simulink model "model"  (R2014a)
(part 6 of 6)

  Pärnu_Jaagupi_haruliin_CN_35450914_110000_CN_35450919_110000/RConn3 -- T_35450919_110000;35000;10000_Audru_alajaam/LConn3 -- bus19/LConn1
  T_35394600_110000;35000;10000_Otepää_alajaam/LConn1 -- _CN_35394600_110000_CN_35420119_110000/LConn1
  T_35394600_110000;35000;10000_Otepää_alajaam/LConn2 -- _CN_35394600_110000_CN_35420119_110000/LConn2
  _CN_35394600_110000_CN_35420119_110000/LConn3 -- T_35394600_110000;35000;10000_Otepää_alajaam/LConn3 -- bus20/LConn1
  _CN_35394600_110000_CN_35420119_110000/RConn1 -- T_35420119_110000;15000;400_Elva_alajaam/LConn1 -- Maaritsa_—_Kanepi_110_kV_CN_35445333_110000_CN_35420119_110000/LConn1
  _CN_35394600_110000_CN_35420119_110000/RConn2 -- T_35420119_110000;15000;400_Elva_alajaam/LConn2 -- Maaritsa_—_Kanepi_110_kV_CN_35445333_110000_CN_35420119_110000/LConn2
  _CN_35394600_110000_CN_35420119_110000/RConn3 -- T_35420119_110000;15000;400_Elva_alajaam/LConn3 -- Maaritsa_—_Kanepi_110_kV_CN_35445333_110000_CN_35420119_110000/LConn3 -- bus21/LConn1
  Alutaguse_—_Estonia_Põhja_110_kV_CN_35367472_110000_CN_35594689_110000/LConn1 -- T_35367472_110000;35000;6000_Alutaguse_alajaam/LConn1 -- _CN_35367472_110000_CN_290177759_110000/LConn1 -- _CN_35367472_110000_CN_35451776_110000/LConn1 -- _CN_35367472_110000_CN_35451774_110000/LConn1 -- _CN_35367472_110000_CN_263282453_110000/LConn1 -- Kiikla_—_Alutaguse_110_kV_CN_35367472_110000_CN_263282454_110000/LConn1 -- Kiikla_—_Alutaguse_110_kV_CN_35367472_110000_CN_34920675_110000/RConn1 -- _CN_35367472_110000_CN_205980356_110000/RConn1 -- _CN_35367472_110000_CN_35367491_110000/LConn1 -- Alutaguse_—_Konsu_110_kV_CN_35367472_110000_CN_34903294_110000/LConn1
  Alutaguse_—_Estonia_Põhja_110_kV_CN_35367472_110000_CN_35594689_110000/LConn2 -- T_35367472_110000;35000;6000_Alutaguse_alajaam/LConn2 -- _CN_35367472_110000_CN_290177759_110000/LConn2 -- _CN_35367472_110000_CN_35451776_110000/LConn2 -- _CN_35367472_110000_CN_35451774_110000/LConn2 -- _CN_35367472_110000_CN_263282453_110000/LConn2 -- Kiikla_—_Alutaguse_110_kV_CN_35367472_110000_CN_263282454_110000/LConn2 -- Kiikla_—_Alutaguse_110_kV_CN_35367472_110000_CN_34920675_110000/RConn2 -- _CN_35367472_110000_CN_205980356_110000/RConn2 -- _CN_35367472_110000_CN_35367491_110000/LConn2 -- Alutaguse_—_Konsu_110_kV_CN_35367472_110000_CN_34903294_110000/LConn2
  Alutaguse_—_Estonia_Põhja_110_kV_CN_35367472_110000_CN_35594689_110000/LConn3 -- T_35367472_110000;35000;6000_Alutaguse_alajaam/LConn3 -- _CN_35367472_110000_CN_290177759_110000/LConn3 -- _CN_35367472_110000_CN_35451776_110000/LConn3 -- _CN_35367472_110000_CN_35451774_110000/LConn3 -- _CN_35367472_110000_CN_263282453_110000/LConn3 -- bus22/LConn1 -- Kiikla_—_Alutaguse_110_kV_CN_35367472_110000_CN_263282454_110000/LConn3 -- Kiikla_—_Alutaguse_110_kV_CN_35367472_110000_CN_34920675_110000/RConn3 -- _CN_35367472_110000_CN_205980356_110000/RConn3 -- _CN_35367472_110000_CN_35367491_110000/LConn3 -- Alutaguse_—_Konsu_110_kV_CN_35367472_110000_CN_34903294_110000/LConn3
  T_35594689__/LConn1 -- Alutaguse_—_Estonia_Põhja_110_kV_CN_35367472_110000_CN_35594689_110000/RConn1
  T_35594689__/LConn2 -- Alutaguse_—_Estonia_Põhja_110_kV_CN_35367472_110000_CN_35594689_110000/RConn2
  Alutaguse_—_Estonia_Põhja_110_kV_CN_35367472_110000_CN_35594689_110000/RConn3 -- T_35594689__/LConn3 -- bus23/LConn1
  T_34903294_110000;35000;6000_Konsu_alajaam/LConn1 -- Alutaguse_—_Konsu_110_kV_CN_35367472_110000_CN_34903294_110000/RConn1
  T_34903294_110000;35000;6000_Konsu_alajaam/LConn2 -- Alutaguse_—_Konsu_110_kV_CN_35367472_110000_CN_34903294_110000/RConn2
  Alutaguse_—_Konsu_110_kV_CN_35367472_110000_CN_34903294_110000/RConn3 -- T_34903294_110000;35000;6000_Konsu_alajaam/LConn3 -- bus24/LConn1
  T_263282454_110000;6000_Kiikla_alajaam/LConn1 -- Kiikla_—_Alutaguse_110_kV_CN_35367472_110000_CN_263282454_110000/RConn1
  T_263282454_110000;6000_Kiikla_alajaam/LConn2 -- Kiikla_—_Alutaguse_110_kV_CN_35367472_110000_CN_263282454_110000/RConn2
  Kiikla_—_Alutaguse_110_kV_CN_35367472_110000_CN_263282454_110000/RConn3 -- T_263282454_110000;6000_Kiikla_alajaam/LConn3 -- bus25/LConn1
  _CN_35367472_110000_CN_35367491_110000/RConn1 -- T_35367491_110000;35000;10000;6000_Aidu_alajaam/LConn1 -- Püssi_—_Aidu_110_kV_CN_35367491_110000_CN_34920713_110000/LConn1 -- Püssi_—_Aidu_110_kV_CN_35367491_110000_CN_34920699_110000/LConn1 -- _CN_35367491_110000_CN_35594719_110000/LConn1 -- Püssi_—_Aidu_110_kV_CN_35367491_110000_CN_34920675_110000/RConn1
  _CN_35367472_110000_CN_35367491_110000/RConn2 -- T_35367491_110000;35000;10000;6000_Aidu_alajaam/LConn2 -- Püssi_—_Aidu_110_kV_CN_35367491_110000_CN_34920713_110000/LConn2 -- Püssi_—_Aidu_110_kV_CN_35367491_110000_CN_34920699_110000/LConn2 -- _CN_35367491_110000_CN_35594719_110000/LConn2 -- Püssi_—_Aidu_110_kV_CN_35367491_110000_CN_34920675_110000/RConn2
  _CN_35367472_110000_CN_35367491_110000/RConn3 -- T_35367491_110000;35000;10000;6000_Aidu_alajaam/LConn3 -- Püssi_—_Aidu_110_kV_CN_35367491_110000_CN_34920713_110000/LConn3 -- Püssi_—_Aidu_110_kV_CN_35367491_110000_CN_34920699_110000/LConn3 -- bus26/LConn1 -- _CN_35367491_110000_CN_35594719_110000/LConn3 -- Püssi_—_Aidu_110_kV_CN_35367491_110000_CN_34920675_110000/RConn3
  T_290177759_110000_Illuka_alajaam/LConn1 -- _CN_35367472_110000_CN_290177759_110000/RConn1
  T_290177759_110000_Illuka_alajaam/LConn2 -- _CN_35367472_110000_CN_290177759_110000/RConn2
  _CN_35367472_110000_CN_290177759_110000/RConn3 -- T_290177759_110000_Illuka_alajaam/LConn3 -- bus27/LConn1
  _CN_35367472_110000_CN_35451776_110000/RConn1 -- T_35451776_110000;35000;15000;10000_Mustvee_alajaam/LConn1 -- Saare_—_Mustvee_110_kV_CN_35451776_110000_CN_180118919_110000/LConn1
  _CN_35367472_110000_CN_35451776_110000/RConn2 -- T_35451776_110000;35000;15000;10000_Mustvee_alajaam/LConn2 -- Saare_—_Mustvee_110_kV_CN_35451776_110000_CN_180118919_110000/LConn2
  _CN_35367472_110000_CN_35451776_110000/RConn3 -- T_35451776_110000;35000;15000;10000_Mustvee_alajaam/LConn3 -- Saare_—_Mustvee_110_kV_CN_35451776_110000_CN_180118919_110000/LConn3 -- bus28/LConn1
  _CN_35367472_110000_CN_35451774_110000/RConn1 -- T_35451774_110000;35000;15000;10000_Jõgeva_alajaam/LConn1 -- Jõgeva_—_Põdra_110_kV_CN_263282458_110000_CN_35451774_110000/LConn1
  _CN_35367472_110000_CN_35451774_110000/RConn2 -- T_35451774_110000;35000;15000;10000_Jõgeva_alajaam/LConn2 -- Jõgeva_—_Põdra_110_kV_CN_263282458_110000_CN_35451774_110000/LConn2
  _CN_35367472_110000_CN_35451774_110000/RConn3 -- T_35451774_110000;35000;15000;10000_Jõgeva_alajaam/LConn3 -- Jõgeva_—_Põdra_110_kV_CN_263282458_110000_CN_35451774_110000/LConn3 -- bus29/LConn1
  T_263282453_110000;10000_Kantküla_alajaam/LConn1 -- _CN_35367472_110000_CN_263282453_110000/RConn1
  T_263282453_110000;10000_Kantküla_alajaam/LConn2 -- _CN_35367472_110000_CN_263282453_110000/RConn2
  _CN_35367472_110000_CN_263282453_110000/RConn3 -- T_263282453_110000;10000_Kantküla_alajaam/LConn3 -- bus30/LConn1
  _CN_35022089_110000_CN_35022082_110000/LConn1 -- T_35022089_110000;35000;10000_Sikassaare_alajaam/LConn1 -- _CN_35022089_110000_CN_35022087_110000/LConn1 -- _CN_35022089_110000_CN_35022100_110000/LConn1
  _CN_35022089_110000_CN_35022082_110000/LConn2 -- T_35022089_110000;35000;10000_Sikassaare_alajaam/LConn2 -- _CN_35022089_110000_CN_35022087_110000/LConn2 -- _CN_35022089_110000_CN_35022100_110000/LConn2
  _CN_35022089_110000_CN_35022082_110000/LConn3 -- T_35022089_110000;35000;10000_Sikassaare_alajaam/LConn3 -- _CN_35022089_110000_CN_35022087_110000/LConn3 -- _CN_35022089_110000_CN_35022100_110000/LConn3 -- bus31/LConn1
  T_35022082_110000;10000_Orissaare_alajaam/LConn1 -- _CN_35022089_110000_CN_35022082_110000/RConn1
  T_35022082_110000;10000_Orissaare_alajaam/LConn2 -- _CN_35022089_110000_CN_35022082_110000/RConn2
  _CN_35022089_110000_CN_35022082_110000/RConn3 -- T_35022082_110000;10000_Orissaare_alajaam/LConn3 -- bus32/LConn1
  T_35022087_110000;10000_Valjala_alajaam/LConn1 -- _CN_35022089_110000_CN_35022087_110000/RConn1
  T_35022087_110000;10000_Valjala_alajaam/LConn2 -- _CN_35022089_110000_CN_35022087_110000/RConn2
  _CN_35022089_110000_CN_35022087_110000/RConn3 -- T_35022087_110000;10000_Valjala_alajaam/LConn3 -- bus33/LConn1
  T_35022100_110000;35000;10000_Leisi_alajaam/LConn1 -- _CN_35022089_110000_CN_35022100_110000/RConn1
  T_35022100_110000;35000;10000_Leisi_alajaam/LConn2 -- _CN_35022089_110000_CN_35022100_110000/RConn2
  _CN_35022089_110000_CN_35022100_110000/RConn3 -- T_35022100_110000;35000;10000_Leisi_alajaam/LConn3 -- bus34/LConn1
  T_35367481_110000_Allika_alajaam/LConn1 -- Balti_EJ_—_Allika_110_kV_CN_35367481_110000_CN_34682059_110000/RConn1
  T_35367481_110000_Allika_alajaam/LConn2 -- Balti_EJ_—_Allika_110_kV_CN_35367481_110000_CN_34682059_110000/RConn2
  Balti_EJ_—_Allika_110_kV_CN_35367481_110000_CN_34682059_110000/RConn3 -- T_35367481_110000_Allika_alajaam/LConn3 -- bus35/LConn1
  T_35451772_110000;15000_Suure_Jaani_alajaam/LConn1 -- Paide_—_Türi_—_Vändra_110_kV_CN_35450940_110000_CN_35451772_110000/RConn1
  T_35451772_110000;15000_Suure_Jaani_alajaam/LConn2 -- Paide_—_Türi_—_Vändra_110_kV_CN_35450940_110000_CN_35451772_110000/RConn2
  Paide_—_Türi_—_Vändra_110_kV_CN_35450940_110000_CN_35451772_110000/RConn3 -- T_35451772_110000;15000_Suure_Jaani_alajaam/LConn3 -- bus36/LConn1
  T_35451763_110000;35000;10000_Türi_alajaam/LConn1 -- Paide_—_Türi_—_Vändra_110_kV_CN_35450940_110000_CN_35451763_110000/RConn1
  T_35451763_110000;35000;10000_Türi_alajaam/LConn2 -- Paide_—_Türi_—_Vändra_110_kV_CN_35450940_110000_CN_35451763_110000/RConn2
  Paide_—_Türi_—_Vändra_110_kV_CN_35450940_110000_CN_35451763_110000/RConn3 -- T_35451763_110000;35000;10000_Türi_alajaam/LConn3 -- bus37/LConn1
  Paide_—_Türi_—_Vändra_110_kV_CN_35450940_110000_CN_35343343_110000/RConn1 -- T_35343343_330000;110000;35000;10000_Paide_alajaam/RConn1 -- Paide_—_Rapla_110_kV_CN_35343343_110000_CN_35379710_110000/LConn1 -- L_35343343/LConn1 -- _CN_34903268_110000_CN_35343343_110000/LConn1
  Paide_—_Türi_—_Vändra_110_kV_CN_35450940_110000_CN_35343343_110000/RConn2 -- T_35343343_330000;110000;35000;10000_Paide_alajaam/RConn2 -- Paide_—_Rapla_110_kV_CN_35343343_110000_CN_35379710_110000/LConn2 -- L_35343343/LConn2 -- _CN_34903268_110000_CN_35343343_110000/LConn2
  Paide_—_Türi_—_Vändra_110_kV_CN_35450940_110000_CN_35343343_110000/RConn3 -- T_35343343_330000;110000;35000;10000_Paide_alajaam/RConn3 -- Paide_—_Rapla_110_kV_CN_35343343_110000_CN_35379710_110000/LConn3 -- L_35343343/LConn3 -- bus38/LConn1 -- _CN_34903268_110000_CN_35343343_110000/LConn3
  T_35594719__/LConn1 -- _CN_35367491_110000_CN_35594719_110000/RConn1
  T_35594719__/LConn2 -- _CN_35367491_110000_CN_35594719_110000/RConn2
  _CN_35367491_110000_CN_35594719_110000/RConn3 -- T_35594719__/LConn3 -- bus39/LConn1
  T_34920713_110000;35000;10000_Väike_Maarja_alajaam/LConn1 -- Püssi_—_Aidu_110_kV_CN_35367491_110000_CN_34920713_110000/RConn1
  T_34920713_110000;35000;10000_Väike_Maarja_alajaam/LConn2 -- Püssi_—_Aidu_110_kV_CN_35367491_110000_CN_34920713_110000/RConn2
  Püssi_—_Aidu_110_kV_CN_35367491_110000_CN_34920713_110000/RConn3 -- T_34920713_110000;35000;10000_Väike_Maarja_alajaam/LConn3 -- bus40/LConn1
  Püssi_—_Aidu_110_kV_CN_35367491_110000_CN_34920699_110000/RConn1 -- T_34920699_330000;110000;35000;10000_Rakvere_alajaam/RConn1 -- Tapa_—_Rakvere_110_kV_CN_34920699_110000_CN_35384064_110000/RConn1 -- L_34920699/LConn1 -- _CN_34920702_110000_CN_34920699_110000/LConn1 -- Haljala_haruliin_CN_34920691_110000_CN_34920699_110000/LConn1
  Püssi_—_Aidu_110_kV_CN_35367491_110000_CN_34920699_110000/RConn2 -- T_34920699_330000;110000;35000;10000_Rakvere_alajaam/RConn2 -- Tapa_—_Rakvere_110_kV_CN_34920699_110000_CN_35384064_110000/RConn2 -- L_34920699/LConn2 -- _CN_34920702_110000_CN_34920699_110000/LConn2 -- Haljala_haruliin_CN_34920691_110000_CN_34920699_110000/LConn2
  Püssi_—_Aidu_110_kV_CN_35367491_110000_CN_34920699_110000/RConn3 -- T_34920699_330000;110000;35000;10000_Rakvere_alajaam/RConn3 -- Tapa_—_Rakvere_110_kV_CN_34920699_110000_CN_35384064_110000/RConn3 -- L_34920699/LConn3 -- bus41/LConn1 -- _CN_34920702_110000_CN_34920699_110000/LConn3 -- Haljala_haruliin_CN_34920691_110000_CN_34920699_110000/LConn3
  Kanepi_—_Võru_110_kV_CN_35445333_110000_CN_35445334_110000/LConn1 -- T_35445333__/LConn1 -- Maaritsa_—_Kanepi_110_kV_CN_35445333_110000_CN_35420117_110000/LConn1 -- Maaritsa_—_Kanepi_110_kV_CN_35445333_110000_CN_35420119_110000/RConn1 -- Maaritsa_—_Kanepi_110_kV_CN_35445333_110000_CN_262457166_110000/LConn1 -- Maaritsa_—_Kanepi_110_kV_CN_35445333_110000_CN_34682089_110000/LConn1
  Kanepi_—_Võru_110_kV_CN_35445333_110000_CN_35445334_110000/LConn2 -- T_35445333__/LConn2 -- Maaritsa_—_Kanepi_110_kV_CN_35445333_110000_CN_35420117_110000/LConn2 -- Maaritsa_—_Kanepi_110_kV_CN_35445333_110000_CN_35420119_110000/RConn2 -- Maaritsa_—_Kanepi_110_kV_CN_35445333_110000_CN_262457166_110000/LConn2 -- Maaritsa_—_Kanepi_110_kV_CN_35445333_110000_CN_34682089_110000/LConn2
  Kanepi_—_Võru_110_kV_CN_35445333_110000_CN_35445334_110000/LConn3 -- T_35445333__/LConn3 -- Maaritsa_—_Kanepi_110_kV_CN_35445333_110000_CN_35420117_110000/LConn3 -- Maaritsa_—_Kanepi_110_kV_CN_35445333_110000_CN_35420119_110000/RConn3 -- Maaritsa_—_Kanepi_110_kV_CN_35445333_110000_CN_262457166_110000/LConn3 -- Maaritsa_—_Kanepi_110_kV_CN_35445333_110000_CN_34682089_110000/LConn3 -- bus42/LConn1
  Kanepi_—_Võru_110_kV_CN_35445333_110000_CN_35445334_110000/RConn1 -- T_35445334_110000;35000;10000_Võru_alajaam/LConn1 -- Võru_—_Soo_110_kV_CN_35445334_110000_CN_35445340_110000/LConn1 -- Võru_—_Põlva_110_kV_CN_35445334_110000_CN_35594687_110000/LConn1 -- Võru_—_Põlva_110_kV_CN_35445334_110000_CN_35445343_110000/LConn1 -- _CN_35445334_110000_CN_182242759_110000/LConn1 -- _CN_35445334_110000_CN_34685113_110000/LConn1 -- _CN_35445334_110000_CN_35445335_110000/LConn1 -- _CN_35445334_110000_CN_182774903_110000/LConn1 -- _CN_35445334_110000_CN_263235177_110000/LConn1
  Kanepi_—_Võru_110_kV_CN_35445333_110000_CN_35445334_110000/RConn2 -- T_35445334_110000;35000;10000_Võru_alajaam/LConn2 -- Võru_—_Soo_110_kV_CN_35445334_110000_CN_35445340_110000/LConn2 -- Võru_—_Põlva_110_kV_CN_35445334_110000_CN_35594687_110000/LConn2 -- Võru_—_Põlva_110_kV_CN_35445334_110000_CN_35445343_110000/LConn2 -- _CN_35445334_110000_CN_182242759_110000/LConn2 -- _CN_35445334_110000_CN_34685113_110000/LConn2 -- _CN_35445334_110000_CN_35445335_110000/LConn2 -- _CN_35445334_110000_CN_182774903_110000/LConn2 -- _CN_35445334_110000_CN_263235177_110000/LConn2
  Kanepi_—_Võru_110_kV_CN_35445333_110000_CN_35445334_110000/RConn3 -- T_35445334_110000;35000;10000_Võru_alajaam/LConn3 -- Võru_—_Soo_110_kV_CN_35445334_110000_CN_35445340_110000/LConn3 -- Võru_—_Põlva_110_kV_CN_35445334_110000_CN_35594687_110000/LConn3 -- Võru_—_Põlva_110_kV_CN_35445334_110000_CN_35445343_110000/LConn3 -- _CN_35445334_110000_CN_182242759_110000/LConn3 -- _CN_35445334_110000_CN_34685113_110000/LConn3 -- _CN_35445334_110000_CN_35445335_110000/LConn3 -- _CN_35445334_110000_CN_182774903_110000/LConn3 -- _CN_35445334_110000_CN_263235177_110000/LConn3 -- bus43/LConn1
  T_35420117_110000;10000_Maaritsa_alajaam/LConn1 -- Maaritsa_—_Kanepi_110_kV_CN_35445333_110000_CN_35420117_110000/RConn1
  T_35420117_110000;10000_Maaritsa_alajaam/LConn2 -- Maaritsa_—_Kanepi_110_kV_CN_35445333_110000_CN_35420117_110000/RConn2
  Maaritsa_—_Kanepi_110_kV_CN_35445333_110000_CN_35420117_110000/RConn3 -- T_35420117_110000;10000_Maaritsa_alajaam/LConn3 -- bus44/LConn1
  Maaritsa_—_Kanepi_110_kV_CN_35445333_110000_CN_262457166_110000/RConn1 -- T_262457166_110000;35000;15000;10000_Rõngu_alajaam/LConn1 -- Rõngu_—_Tõrva_110_kV_CN_35445348_110000_CN_262457166_110000/LConn1
  Maaritsa_—_Kanepi_110_kV_CN_35445333_110000_CN_262457166_110000/RConn2 -- T_262457166_110000;35000;15000;10000_Rõngu_alajaam/LConn2 -- Rõngu_—_Tõrva_110_kV_CN_35445348_110000_CN_262457166_110000/LConn2
  Maaritsa_—_Kanepi_110_kV_CN_35445333_110000_CN_262457166_110000/RConn3 -- T_262457166_110000;35000;15000;10000_Rõngu_alajaam/LConn3 -- Rõngu_—_Tõrva_110_kV_CN_35445348_110000_CN_262457166_110000/LConn3 -- bus45/LConn1
  Maaritsa_—_Kanepi_110_kV_CN_35445333_110000_CN_34682089_110000/RConn1 -- T_34682089_330000;110000;35000;15000;10000_Tartu_alajaam/RConn1 -- Voldi_haruliin_CN_101153487_110000_CN_34682089_110000/LConn1 -- Tartu_—_Anne_&_Tartu_—_Tööstuse_110_kV_CN_34682089_110000_CN_30228363_110000/LConn1 -- Tartu_—_Emajõe_110_kV_CN_34682089_110000_CN_30222062_110000/LConn1 -- L_34682089/LConn1
  Maaritsa_—_Kanepi_110_kV_CN_35445333_110000_CN_34682089_110000/RConn2 -- T_34682089_330000;110000;35000;15000;10000_Tartu_alajaam/RConn2 -- Voldi_haruliin_CN_101153487_110000_CN_34682089_110000/LConn2 -- Tartu_—_Anne_&_Tartu_—_Tööstuse_110_kV_CN_34682089_110000_CN_30228363_110000/LConn2 -- Tartu_—_Emajõe_110_kV_CN_34682089_110000_CN_30222062_110000/LConn2 -- L_34682089/LConn2
  Maaritsa_—_Kanepi_110_kV_CN_35445333_110000_CN_34682089_110000/RConn3 -- T_34682089_330000;110000;35000;15000;10000_Tartu_alajaam/RConn3 -- Voldi_haruliin_CN_101153487_110000_CN_34682089_110000/LConn3 -- Tartu_—_Anne_&_Tartu_—_Tööstuse_110_kV_CN_34682089_110000_CN_30228363_110000/LConn3 -- Tartu_—_Emajõe_110_kV_CN_34682089_110000_CN_30222062_110000/LConn3 -- L_34682089/LConn3 -- bus46/LConn1
  T_35445340_110000;10000_Soo_alajaam/LConn1 -- Võru_—_Soo_110_kV_CN_35445334_110000_CN_35445340_110000/RConn1
  T_35445340_110000;10000_Soo_alajaam/LConn2 -- Võru_—_Soo_110_kV_CN_35445334_110000_CN_35445340_110000/RConn2
  Võru_—_Soo_110_kV_CN_35445334_110000_CN_35445340_110000/RConn3 -- T_35445340_110000;10000_Soo_alajaam/LConn3 -- bus47/LConn1
  T_35594687_110000;10000_Ruusa_alajaam/LConn1 -- Võru_—_Põlva_110_kV_CN_35445334_110000_CN_35594687_110000/RConn1
  T_35594687_110000;10000_Ruusa_alajaam/LConn2 -- Võru_—_Põlva_110_kV_CN_35445334_110000_CN_35594687_110000/RConn2
  Võru_—_Põlva_110_kV_CN_35445334_110000_CN_35594687_110000/RConn3 -- T_35594687_110000;10000_Ruusa_alajaam/LConn3 -- bus48/LConn1
  Võru_—_Põlva_110_kV_CN_35445334_110000_CN_35445343_110000/RConn1 -- T_35445343__Põlva_alajaam/LConn1 -- Kuuste_—_Põlva_110_kV_CN_35445343_110000_CN_35445346_110000/LConn1
  Võru_—_Põlva_110_kV_CN_35445334_110000_CN_35445343_110000/RConn2 -- T_35445343__Põlva_alajaam/LConn2 -- Kuuste_—_Põlva_110_kV_CN_35445343_110000_CN_35445346_110000/LConn2
  Võru_—_Põlva_110_kV_CN_35445334_110000_CN_35445343_110000/RConn3 -- T_35445343__Põlva_alajaam/LConn3 -- Kuuste_—_Põlva_110_kV_CN_35445343_110000_CN_35445346_110000/LConn3 -- bus49/LConn1
  _CN_35445334_110000_CN_182242759_110000/RConn1 -- T_182242759_110000;10000_Rõuge_alajaam/LConn1 -- _CN_263253461_110000_CN_182242759_110000/LConn1
  _CN_35445334_110000_CN_182242759_110000/RConn2 -- T_182242759_110000;10000_Rõuge_alajaam/LConn2 -- _CN_263253461_110000_CN_182242759_110000/LConn2
  _CN_35445334_110000_CN_182242759_110000/RConn3 -- T_182242759_110000;10000_Rõuge_alajaam/LConn3 -- _CN_263253461_110000_CN_182242759_110000/LConn3 -- bus50/LConn1
  _CN_35445334_110000_CN_34685113_110000/RConn1 -- T_34685113_330000;110000;35000;10000_Tsinguliina_alajaam/RConn1 -- Tsirguliina_—_Tõrva_110_kV_CN_35445348_110000_CN_34685113_110000/LConn1 -- _CN_34685113_110000_CN_35450869_110000/LConn1 -- L_34685113/LConn1
  _CN_35445334_110000_CN_34685113_110000/RConn2 -- T_34685113_330000;110000;35000;10000_Tsinguliina_alajaam/RConn2 -- Tsirguliina_—_Tõrva_110_kV_CN_35445348_110000_CN_34685113_110000/LConn2 -- _CN_34685113_110000_CN_35450869_110000/LConn2 -- L_34685113/LConn2
  _CN_35445334_110000_CN_34685113_110000/RConn3 -- T_34685113_330000;110000;35000;10000_Tsinguliina_alajaam/RConn3 -- Tsirguliina_—_Tõrva_110_kV_CN_35445348_110000_CN_34685113_110000/LConn3 -- _CN_34685113_110000_CN_35450869_110000/LConn3 -- L_34685113/LConn3 -- bus51/LConn1
  T_35445335_110000;35000;10000_Mõniste_alajaam/LConn1 -- _CN_35445334_110000_CN_35445335_110000/RConn1
  T_35445335_110000;35000;10000_Mõniste_alajaam/LConn2 -- _CN_35445334_110000_CN_35445335_110000/RConn2
  _CN_35445334_110000_CN_35445335_110000/RConn3 -- T_35445335_110000;35000;10000_Mõniste_alajaam/LConn3 -- bus52/LConn1
  T_182774903_110000;10000_Linda_alajaam/LConn1 -- _CN_35445334_110000_CN_182774903_110000/RConn1
  T_182774903_110000;10000_Linda_alajaam/LConn2 -- _CN_35445334_110000_CN_182774903_110000/RConn2
  _CN_35445334_110000_CN_182774903_110000/RConn3 -- T_182774903_110000;10000_Linda_alajaam/LConn3 -- bus53/LConn1
  T_263235177_110000;10000_Sõmerpalu_alajaam/LConn1 -- _CN_35445334_110000_CN_263235177_110000/RConn1
  T_263235177_110000;10000_Sõmerpalu_alajaam/LConn2 -- _CN_35445334_110000_CN_263235177_110000/RConn2
  _CN_35445334_110000_CN_263235177_110000/RConn3 -- T_263235177_110000;10000_Sõmerpalu_alajaam/LConn3 -- bus54/LConn1
  Kuuste_—_Põlva_110_kV_CN_35445343_110000_CN_35445346_110000/RConn1 -- T_35445346_110000;10000_Kuuste_alajaam/LConn1 -- Anne_—_Kuuste_110_kV_CN_35445346_110000_CN_30228363_110000/LConn1 -- Anne_—_Kuuste_110_kV_CN_35445346_110000_CN_35594688_110000/LConn1
  Kuuste_—_Põlva_110_kV_CN_35445343_110000_CN_35445346_110000/RConn2 -- T_35445346_110000;10000_Kuuste_alajaam/LConn2 -- Anne_—_Kuuste_110_kV_CN_35445346_110000_CN_30228363_110000/LConn2 -- Anne_—_Kuuste_110_kV_CN_35445346_110000_CN_35594688_110000/LConn2
  Kuuste_—_Põlva_110_kV_CN_35445343_110000_CN_35445346_110000/RConn3 -- T_35445346_110000;10000_Kuuste_alajaam/LConn3 -- Anne_—_Kuuste_110_kV_CN_35445346_110000_CN_30228363_110000/LConn3 -- Anne_—_Kuuste_110_kV_CN_35445346_110000_CN_35594688_110000/LConn3 -- bus55/LConn1
  Anne_—_Kuuste_110_kV_CN_35445346_110000_CN_30228363_110000/RConn1 -- T_30228363_110000;35000;15000;10000_Anne_alajaam/LConn1 -- Tartu_—_Anne_&_Tartu_—_Tööstuse_110_kV_CN_34682089_110000_CN_30228363_110000/RConn1
  Anne_—_Kuuste_110_kV_CN_35445346_110000_CN_30228363_110000/RConn2 -- T_30228363_110000;35000;15000;10000_Anne_alajaam/LConn2 -- Tartu_—_Anne_&_Tartu_—_Tööstuse_110_kV_CN_34682089_110000_CN_30228363_110000/RConn2
  Anne_—_Kuuste_110_kV_CN_35445346_110000_CN_30228363_110000/RConn3 -- T_30228363_110000;35000;15000;10000_Anne_alajaam/LConn3 -- Tartu_—_Anne_&_Tartu_—_Tööstuse_110_kV_CN_34682089_110000_CN_30228363_110000/RConn3 -- bus56/LConn1
  T_35594688_110000;15000_Alatskivi_alajaam/LConn1 -- Anne_—_Kuuste_110_kV_CN_35445346_110000_CN_35594688_110000/RConn1
  T_35594688_110000;15000_Alatskivi_alajaam/LConn2 -- Anne_—_Kuuste_110_kV_CN_35445346_110000_CN_35594688_110000/RConn2
  Anne_—_Kuuste_110_kV_CN_35445346_110000_CN_35594688_110000/RConn3 -- T_35594688_110000;15000_Alatskivi_alajaam/LConn3 -- bus57/LConn1
  Rõngu_—_Tõrva_110_kV_CN_35445348_110000_CN_262457166_110000/RConn1 -- T_35445348_110000;15000_Tõrva_alajaam/LConn1 -- Tõrva_—_Abja_110_kV_CN_35445348_110000_CN_35450872_110000/LConn1 -- Tsirguliina_—_Tõrva_110_kV_CN_35445348_110000_CN_34685113_110000/RConn1 -- Tsirguliina_—_Tõrva_110_kV_CN_35445348_110000_CN_35450869_110000/LConn1
  Rõngu_—_Tõrva_110_kV_CN_35445348_110000_CN_262457166_110000/RConn2 -- T_35445348_110000;15000_Tõrva_alajaam/LConn2 -- Tõrva_—_Abja_110_kV_CN_35445348_110000_CN_35450872_110000/LConn2 -- Tsirguliina_—_Tõrva_110_kV_CN_35445348_110000_CN_34685113_110000/RConn2 -- Tsirguliina_—_Tõrva_110_kV_CN_35445348_110000_CN_35450869_110000/LConn2
  Rõngu_—_Tõrva_110_kV_CN_35445348_110000_CN_262457166_110000/RConn3 -- T_35445348_110000;15000_Tõrva_alajaam/LConn3 -- Tõrva_—_Abja_110_kV_CN_35445348_110000_CN_35450872_110000/LConn3 -- Tsirguliina_—_Tõrva_110_kV_CN_35445348_110000_CN_34685113_110000/RConn3 -- Tsirguliina_—_Tõrva_110_kV_CN_35445348_110000_CN_35450869_110000/LConn3 -- bus58/LConn1
  T_35450872_110000;15000_Abja_alajaam/LConn1 -- Tõrva_—_Abja_110_kV_CN_35445348_110000_CN_35450872_110000/RConn1
  T_35450872_110000;15000_Abja_alajaam/LConn2 -- Tõrva_—_Abja_110_kV_CN_35445348_110000_CN_35450872_110000/RConn2
  Tõrva_—_Abja_110_kV_CN_35445348_110000_CN_35450872_110000/RConn3 -- T_35450872_110000;15000_Abja_alajaam/LConn3 -- bus59/LConn1
  Tsirguliina_—_Tõrva_110_kV_CN_35445348_110000_CN_35450869_110000/RConn1 -- T_35450869_110000;10000_Valga_alajaam/LConn1 -- _CN_34685113_110000_CN_35450869_110000/RConn1
  Tsirguliina_—_Tõrva_110_kV_CN_35445348_110000_CN_35450869_110000/RConn2 -- T_35450869_110000;10000_Valga_alajaam/LConn2 -- _CN_34685113_110000_CN_35450869_110000/RConn2
  Tsirguliina_—_Tõrva_110_kV_CN_35445348_110000_CN_35450869_110000/RConn3 -- T_35450869_110000;10000_Valga_alajaam/LConn3 -- _CN_34685113_110000_CN_35450869_110000/RConn3 -- bus60/LConn1
  Kiisa_—_Keila_110_kV_CN_34935436_110000_CN_262229346_110000/LConn1 -- T_34935436_330000;220000;110000;35000;10000_Kiisa_alajaam/RConn1 -- _CN_34935436_110000_CN_265791084_110000/LConn1 -- L_34935436/LConn1 -- Kiisa_—_Järve_110_kV_CN_34935436_110000_CN_34968246_110000/LConn1 -- Kiisa_—_Järve_110_kV_CN_34935436_110000_CN_34968285_110000/LConn1 -- Kiisa_—_Ellamaa_CN_34935436_110000_CN_35379710_110000/LConn1 -- Kiisa_—_Ellamaa_CN_34935436_110000_CN_34988535_110000/LConn1 -- Kiisa_—_Ellamaa_CN_34935436_110000_CN_34988502_110000/LConn1 -- Harku_—_Kiisa_110_kV_CN_34935436_110000_CN_34968224_110000/LConn1 -- Kiisa_—_Laagri_110_kV_CN_34935436_110000_CN_34988471_110000/LConn1 -- Kiisa_—_Laagri_110_kV_CN_34935436_110000_CN_34935452_110000/LConn1
  Kiisa_—_Keila_110_kV_CN_34935436_110000_CN_262229346_110000/LConn2 -- T_34935436_330000;220000;110000;35000;10000_Kiisa_alajaam/RConn2 -- _CN_34935436_110000_CN_265791084_110000/LConn2 -- L_34935436/LConn2 -- Kiisa_—_Järve_110_kV_CN_34935436_110000_CN_34968246_110000/LConn2 -- Kiisa_—_Järve_110_kV_CN_34935436_110000_CN_34968285_110000/LConn2 -- Kiisa_—_Ellamaa_CN_34935436_110000_CN_35379710_110000/LConn2 -- Kiisa_—_Ellamaa_CN_34935436_110000_CN_34988535_110000/LConn2 -- Kiisa_—_Ellamaa_CN_34935436_110000_CN_34988502_110000/LConn2 -- Harku_—_Kiisa_110_kV_CN_34935436_110000_CN_34968224_110000/LConn2 -- Kiisa_—_Laagri_110_kV_CN_34935436_110000_CN_34988471_110000/LConn2 -- Kiisa_—_Laagri_110_kV_CN_34935436_110000_CN_34935452_110000/LConn2
  Kiisa_—_Keila_110_kV_CN_34935436_110000_CN_262229346_110000/LConn3 -- T_34935436_330000;220000;110000;35000;10000_Kiisa_alajaam/RConn3 -- _CN_34935436_110000_CN_265791084_110000/LConn3 -- L_34935436/LConn3 -- bus61/LConn1 -- Kiisa_—_Järve_110_kV_CN_34935436_110000_CN_34968246_110000/LConn3 -- Kiisa_—_Järve_110_kV_CN_34935436_110000_CN_34968285_110000/LConn3 -- Kiisa_—_Ellamaa_CN_34935436_110000_CN_35379710_110000/LConn3 -- Kiisa_—_Ellamaa_CN_34935436_110000_CN_34988535_110000/LConn3 -- Kiisa_—_Ellamaa_CN_34935436_110000_CN_34988502_110000/LConn3 -- Harku_—_Kiisa_110_kV_CN_34935436_110000_CN_34968224_110000/LConn3 -- Kiisa_—_Laagri_110_kV_CN_34935436_110000_CN_34988471_110000/LConn3 -- Kiisa_—_Laagri_110_kV_CN_34935436_110000_CN_34935452_110000/LConn3
  Kiisa_—_Keila_110_kV_CN_34935436_110000_CN_262229346_110000/RConn1 -- T_262229346_110000;35000;10000_Keila_alajaam/LConn1 -- Keila_—_Paldiski_110_kV_CN_35550404_110000_CN_262229346_110000/LConn1 -- Keila_—_Rummu_110_kV_CN_262229346_110000_CN_34988486_110000/LConn1 -- Harku_—_Keila_110_kV_CN_34968224_110000_CN_262229346_110000/LConn1
  Kiisa_—_Keila_110_kV_CN_34935436_110000_CN_262229346_110000/RConn2 -- T_262229346_110000;35000;10000_Keila_alajaam/LConn2 -- Keila_—_Paldiski_110_kV_CN_35550404_110000_CN_262229346_110000/LConn2 -- Keila_—_Rummu_110_kV_CN_262229346_110000_CN_34988486_110000/LConn2 -- Harku_—_Keila_110_kV_CN_34968224_110000_CN_262229346_110000/LConn2
  Kiisa_—_Keila_110_kV_CN_34935436_110000_CN_262229346_110000/RConn3 -- T_262229346_110000;35000;10000_Keila_alajaam/LConn3 -- Keila_—_Paldiski_110_kV_CN_35550404_110000_CN_262229346_110000/LConn3 -- Keila_—_Rummu_110_kV_CN_262229346_110000_CN_34988486_110000/LConn3 -- bus62/LConn1 -- Harku_—_Keila_110_kV_CN_34968224_110000_CN_262229346_110000/LConn3
  Kiisa_—_Järve_110_kV_CN_34935436_110000_CN_34968246_110000/RConn1 -- T_34968246_110000;10000;6000_Järve_alajaam/LConn1 -- Järve_—_Ülemiste_110_kV_CN_34968246_110000_CN_34968248_110000/LConn1 -- Iru_—_Järve_&_Järveküla_—_Järve_110_kV_CN_34968246_110000_CN_34968251_110000/LConn1 -- Iru_—_Järve_&_Järveküla_—_Järve_110_kV_CN_34968246_110000_CN_72668114_110000/LConn1
  Kiisa_—_Järve_110_kV_CN_34935436_110000_CN_34968246_110000/RConn2 -- T_34968246_110000;10000;6000_Järve_alajaam/LConn2 -- Järve_—_Ülemiste_110_kV_CN_34968246_110000_CN_34968248_110000/LConn2 -- Iru_—_Järve_&_Järveküla_—_Järve_110_kV_CN_34968246_110000_CN_34968251_110000/LConn2 -- Iru_—_Järve_&_Järveküla_—_Järve_110_kV_CN_34968246_110000_CN_72668114_110000/LConn2
  Kiisa_—_Järve_110_kV_CN_34935436_110000_CN_34968246_110000/RConn3 -- T_34968246_110000;10000;6000_Järve_alajaam/LConn3 -- Järve_—_Ülemiste_110_kV_CN_34968246_110000_CN_34968248_110000/LConn3 -- Iru_—_Järve_&_Järveküla_—_Järve_110_kV_CN_34968246_110000_CN_34968251_110000/LConn3 -- Iru_—_Järve_&_Järveküla_—_Järve_110_kV_CN_34968246_110000_CN_72668114_110000/LConn3 -- bus63/LConn1
  Kiisa_—_Järve_110_kV_CN_34935436_110000_CN_34968285_110000/RConn1 -- T_34968285_110000;10000_Jüri_alajaam/LConn1 -- Aruküla_—_Jüri_110_kV_CN_34968285_110000_CN_204914596_110000/RConn1
  Kiisa_—_Järve_110_kV_CN_34935436_110000_CN_34968285_110000/RConn2 -- T_34968285_110000;10000_Jüri_alajaam/LConn2 -- Aruküla_—_Jüri_110_kV_CN_34968285_110000_CN_204914596_110000/RConn2
  Kiisa_—_Järve_110_kV_CN_34935436_110000_CN_34968285_110000/RConn3 -- T_34968285_110000;10000_Jüri_alajaam/LConn3 -- Aruküla_—_Jüri_110_kV_CN_34968285_110000_CN_204914596_110000/RConn3 -- bus64/LConn1
  Kiisa_—_Ellamaa_CN_34935436_110000_CN_35379710_110000/RConn1 -- T_35379710_110000;10000_Kohila_alajaam/LConn1 -- Paide_—_Rapla_110_kV_CN_35343343_110000_CN_35379710_110000/RConn1
  Kiisa_—_Ellamaa_CN_34935436_110000_CN_35379710_110000/RConn2 -- T_35379710_110000;10000_Kohila_alajaam/LConn2 -- Paide_—_Rapla_110_kV_CN_35343343_110000_CN_35379710_110000/RConn2
  Kiisa_—_Ellamaa_CN_34935436_110000_CN_35379710_110000/RConn3 -- T_35379710_110000;10000_Kohila_alajaam/LConn3 -- Paide_—_Rapla_110_kV_CN_35343343_110000_CN_35379710_110000/RConn3 -- bus65/LConn1
  T_34988535_110000;35000;10000;6000_Ellamaa_alajaam/LConn1 -- Kiisa_—_Ellamaa_CN_34935436_110000_CN_34988535_110000/RConn1
  T_34988535_110000;35000;10000;6000_Ellamaa_alajaam/LConn2 -- Kiisa_—_Ellamaa_CN_34935436_110000_CN_34988535_110000/RConn2
  Kiisa_—_Ellamaa_CN_34935436_110000_CN_34988535_110000/RConn3 -- T_34988535_110000;35000;10000;6000_Ellamaa_alajaam/LConn3 -- bus66/LConn1
  Kiisa_—_Ellamaa_CN_34935436_110000_CN_34988502_110000/RConn1 -- T_34988502_110000;35000;10000_Risti_alajaam/LConn1 -- Lihula_—_Vigala_110_kV_CN_262755193_110000_CN_34988502_110000/LConn1
  Kiisa_—_Ellamaa_CN_34935436_110000_CN_34988502_110000/RConn2 -- T_34988502_110000;35000;10000_Risti_alajaam/LConn2 -- Lihula_—_Vigala_110_kV_CN_262755193_110000_CN_34988502_110000/LConn2
  Kiisa_—_Ellamaa_CN_34935436_110000_CN_34988502_110000/RConn3 -- T_34988502_110000;35000;10000_Risti_alajaam/LConn3 -- Lihula_—_Vigala_110_kV_CN_262755193_110000_CN_34988502_110000/LConn3 -- bus67/LConn1
  Harku_—_Kiisa_110_kV_CN_34935436_110000_CN_34968224_110000/RConn1 -- T_34968224_330000;110000;20000_Harku_ajajaam/RConn1 -- Harku_—_Veskimetsa_110_kV_CN_34968224_110000_CN_99350295_110000/LConn1 -- _CN_34968224_110000_CN_99369449_110000/LConn1 -- Harku_—_Keila_110_kV_CN_34968224_110000_CN_262229346_110000/RConn1 -- Harku_—_Keila_110_kV_CN_34968224_110000_CN_34988480_110000/LConn1 -- L_34968224/LConn1
  Harku_—_Kiisa_110_kV_CN_34935436_110000_CN_34968224_110000/RConn2 -- T_34968224_330000;110000;20000_Harku_ajajaam/RConn2 -- Harku_—_Veskimetsa_110_kV_CN_34968224_110000_CN_99350295_110000/LConn2 -- _CN_34968224_110000_CN_99369449_110000/LConn2 -- Harku_—_Keila_110_kV_CN_34968224_110000_CN_262229346_110000/RConn2 -- Harku_—_Keila_110_kV_CN_34968224_110000_CN_34988480_110000/LConn2 -- L_34968224/LConn2
  Harku_—_Kiisa_110_kV_CN_34935436_110000_CN_34968224_110000/RConn3 -- T_34968224_330000;110000;20000_Harku_ajajaam/RConn3 -- Harku_—_Veskimetsa_110_kV_CN_34968224_110000_CN_99350295_110000/LConn3 -- _CN_34968224_110000_CN_99369449_110000/LConn3 -- Harku_—_Keila_110_kV_CN_34968224_110000_CN_262229346_110000/RConn3 -- Harku_—_Keila_110_kV_CN_34968224_110000_CN_34988480_110000/LConn3 -- L_34968224/LConn3 -- bus68/LConn1
  T_34988471_110000;10000_Topi_alajaam/LConn1 -- Kiisa_—_Laagri_110_kV_CN_34935436_110000_CN_34988471_110000/RConn1
  T_34988471_110000;10000_Topi_alajaam/LConn2 -- Kiisa_—_Laagri_110_kV_CN_34935436_110000_CN_34988471_110000/RConn2
  Kiisa_—_Laagri_110_kV_CN_34935436_110000_CN_34988471_110000/RConn3 -- T_34988471_110000;10000_Topi_alajaam/LConn3 -- bus69/LConn1
  T_34935452_110000;35000;10000_Laagri_alajaam/LConn1 -- Kiisa_—_Laagri_110_kV_CN_34935436_110000_CN_34935452_110000/RConn1
  T_34935452_110000;35000;10000_Laagri_alajaam/LConn2 -- Kiisa_—_Laagri_110_kV_CN_34935436_110000_CN_34935452_110000/RConn2
  Kiisa_—_Laagri_110_kV_CN_34935436_110000_CN_34935452_110000/RConn3 -- T_34935452_110000;35000;10000_Laagri_alajaam/LConn3 -- bus70/LConn1
  _CN_34935436_110000_CN_265791084_110000/RConn1 -- G_265791084_Kiisa_AREJ/RConn1 -- _CN_34935436_330000_CN_265791084_110000/LConn1
  _CN_34935436_110000_CN_265791084_110000/RConn2 -- G_265791084_Kiisa_AREJ/RConn2 -- _CN_34935436_330000_CN_265791084_110000/LConn2
  _CN_34935436_110000_CN_265791084_110000/RConn3 -- G_265791084_Kiisa_AREJ/RConn3 -- _CN_34935436_330000_CN_265791084_110000/LConn3 -- bus71/LConn1
  T_34920702_110000;35000;10000_Rakvere_Põhja_alajaam/LConn1 -- _CN_34920702_110000_CN_34920699_110000/RConn1
  T_34920702_110000;35000;10000_Rakvere_Põhja_alajaam/LConn2 -- _CN_34920702_110000_CN_34920699_110000/RConn2
  _CN_34920702_110000_CN_34920699_110000/RConn3 -- T_34920702_110000;35000;10000_Rakvere_Põhja_alajaam/LConn3 -- bus72/LConn1
  T_29595798_110000;35000;10000_Loo_alajaam/LConn1 -- _CN_29595798_110000_CN_204914596_110000/RConn1
  T_29595798_110000;35000;10000_Loo_alajaam/LConn2 -- _CN_29595798_110000_CN_204914596_110000/RConn2
  _CN_29595798_110000_CN_204914596_110000/RConn3 -- T_29595798_110000;35000;10000_Loo_alajaam/LConn3 -- bus73/LConn1
  Harku_—_Veskimetsa_110_kV_CN_34968224_110000_CN_99350295_110000/RConn1 -- T_99350295_110000;35000;10000;6000_Veskimetsa_alajaam/LConn1 -- Kopli_—_Paljassaare_110_kV_CN_34968238_110000_CN_99350295_110000/LConn1
  Harku_—_Veskimetsa_110_kV_CN_34968224_110000_CN_99350295_110000/RConn2 -- T_99350295_110000;35000;10000;6000_Veskimetsa_alajaam/LConn2 -- Kopli_—_Paljassaare_110_kV_CN_34968238_110000_CN_99350295_110000/LConn2
  Harku_—_Veskimetsa_110_kV_CN_34968224_110000_CN_99350295_110000/RConn3 -- T_99350295_110000;35000;10000;6000_Veskimetsa_alajaam/LConn3 -- Kopli_—_Paljassaare_110_kV_CN_34968238_110000_CN_99350295_110000/LConn3 -- bus74/LConn1
  T_99369449__Kadaka_alajaam/LConn1 -- _CN_34968224_110000_CN_99369449_110000/RConn1
  T_99369449__Kadaka_alajaam/LConn2 -- _CN_34968224_110000_CN_99369449_110000/RConn2
  _CN_34968224_110000_CN_99369449_110000/RConn3 -- T_99369449__Kadaka_alajaam/LConn3 -- bus75/LConn1
  T_34988480_110000;10000_Tabasalu_alajaam/LConn1 -- Harku_—_Keila_110_kV_CN_34968224_110000_CN_34988480_110000/RConn1
  T_34988480_110000;10000_Tabasalu_alajaam/LConn2 -- Harku_—_Keila_110_kV_CN_34968224_110000_CN_34988480_110000/RConn2
  Harku_—_Keila_110_kV_CN_34968224_110000_CN_34988480_110000/RConn3 -- T_34988480_110000;10000_Tabasalu_alajaam/LConn3 -- bus76/LConn1
  Kopli_—_Paljassaare_110_kV_CN_34968238_110000_CN_34968239_110000/LConn1 -- T_34968238_110000;35000;6000_Kopli_alajaam/LConn1 -- Kopli_—_Paljassaare_110_kV_CN_34968238_110000_CN_85487602_110000/LConn1 -- Kopli_—_Paljassaare_110_kV_CN_34968238_110000_CN_99350295_110000/RConn1
  Kopli_—_Paljassaare_110_kV_CN_34968238_110000_CN_34968239_110000/LConn2 -- T_34968238_110000;35000;6000_Kopli_alajaam/LConn2 -- Kopli_—_Paljassaare_110_kV_CN_34968238_110000_CN_85487602_110000/LConn2 -- Kopli_—_Paljassaare_110_kV_CN_34968238_110000_CN_99350295_110000/RConn2
  Kopli_—_Paljassaare_110_kV_CN_34968238_110000_CN_34968239_110000/LConn3 -- T_34968238_110000;35000;6000_Kopli_alajaam/LConn3 -- Kopli_—_Paljassaare_110_kV_CN_34968238_110000_CN_85487602_110000/LConn3 -- Kopli_—_Paljassaare_110_kV_CN_34968238_110000_CN_99350295_110000/RConn3 -- bus77/LConn1
  T_34968239_110000;6000_Paljassaare_alajaam/LConn1 -- Kopli_—_Paljassaare_110_kV_CN_34968238_110000_CN_34968239_110000/RConn1
  T_34968239_110000;6000_Paljassaare_alajaam/LConn2 -- Kopli_—_Paljassaare_110_kV_CN_34968238_110000_CN_34968239_110000/RConn2
  Kopli_—_Paljassaare_110_kV_CN_34968238_110000_CN_34968239_110000/RConn3 -- T_34968239_110000;6000_Paljassaare_alajaam/LConn3 -- bus78/LConn1
  T_85487602_110000;6000_Uus_Volta_alajaam/LConn1 -- Kopli_—_Paljassaare_110_kV_CN_34968238_110000_CN_85487602_110000/RConn1
  T_85487602_110000;6000_Uus_Volta_alajaam/LConn2 -- Kopli_—_Paljassaare_110_kV_CN_34968238_110000_CN_85487602_110000/RConn2
  Kopli_—_Paljassaare_110_kV_CN_34968238_110000_CN_85487602_110000/RConn3 -- T_85487602_110000;6000_Uus_Volta_alajaam/LConn3 -- bus79/LConn1
  Järve_—_Ülemiste_110_kV_CN_34968246_110000_CN_34968248_110000/RConn1 -- T_34968248_110000;35000;6000_Ülemiste_alajaam/LConn1 -- Lasnamäe_—_Ülemiste_110_kV_CN_34968248_110000_CN_34968269_110000/LConn1
  Järve_—_Ülemiste_110_kV_CN_34968246_110000_CN_34968248_110000/RConn2 -- T_34968248_110000;35000;6000_Ülemiste_alajaam/LConn2 -- Lasnamäe_—_Ülemiste_110_kV_CN_34968248_110000_CN_34968269_110000/LConn2
  Järve_—_Ülemiste_110_kV_CN_34968246_110000_CN_34968248_110000/RConn3 -- T_34968248_110000;35000;6000_Ülemiste_alajaam/LConn3 -- Lasnamäe_—_Ülemiste_110_kV_CN_34968248_110000_CN_34968269_110000/LConn3 -- bus80/LConn1
  T_34968251_110000;20000_Järveküla_alajaam/LConn1 -- Iru_—_Järve_&_Järveküla_—_Järve_110_kV_CN_34968246_110000_CN_34968251_110000/RConn1
  T_34968251_110000;20000_Järveküla_alajaam/LConn2 -- Iru_—_Järve_&_Järveküla_—_Järve_110_kV_CN_34968246_110000_CN_34968251_110000/RConn2
  Iru_—_Järve_&_Järveküla_—_Järve_110_kV_CN_34968246_110000_CN_34968251_110000/RConn3 -- T_34968251_110000;20000_Järveküla_alajaam/LConn3 -- bus81/LConn1
  Iru_—_Järve_&_Järveküla_—_Järve_110_kV_CN_34968246_110000_CN_72668114_110000/RConn1 -- T_72668114_110000;10000_Iru_alajaam/LConn1 -- Iru_—_Kallavere_110_kV_CN_72668114_110000_CN_29979106_110000/LConn1 -- _CN_34968269_110000_CN_72668114_110000/LConn1
  Iru_—_Järve_&_Järveküla_—_Järve_110_kV_CN_34968246_110000_CN_72668114_110000/RConn2 -- T_72668114_110000;10000_Iru_alajaam/LConn2 -- Iru_—_Kallavere_110_kV_CN_72668114_110000_CN_29979106_110000/LConn2 -- _CN_34968269_110000_CN_72668114_110000/LConn2
  Iru_—_Järve_&_Järveküla_—_Järve_110_kV_CN_34968246_110000_CN_72668114_110000/RConn3 -- T_72668114_110000;10000_Iru_alajaam/LConn3 -- Iru_—_Kallavere_110_kV_CN_72668114_110000_CN_29979106_110000/LConn3 -- bus82/LConn1 -- _CN_34968269_110000_CN_72668114_110000/LConn3
  Lasnamäe_—_Ülemiste_110_kV_CN_34968248_110000_CN_34968269_110000/RConn1 -- T_34968269_110000;10000;6000_Lasnamäe_alajaam/LConn1 -- _CN_34968269_110000_CN_72668114_110000/RConn1 -- _CN_34968269_110000_CN_34968270_110000/LConn1
  Lasnamäe_—_Ülemiste_110_kV_CN_34968248_110000_CN_34968269_110000/RConn2 -- T_34968269_110000;10000;6000_Lasnamäe_alajaam/LConn2 -- _CN_34968269_110000_CN_72668114_110000/RConn2 -- _CN_34968269_110000_CN_34968270_110000/LConn2
  Lasnamäe_—_Ülemiste_110_kV_CN_34968248_110000_CN_34968269_110000/RConn3 -- T_34968269_110000;10000;6000_Lasnamäe_alajaam/LConn3 -- _CN_34968269_110000_CN_72668114_110000/RConn3 -- _CN_34968269_110000_CN_34968270_110000/LConn3 -- bus83/LConn1
  T_35550404_110000;35000;10000_Paldiski_alajaam/LConn1 -- Keila_—_Paldiski_110_kV_CN_35550404_110000_CN_262229346_110000/RConn1
  T_35550404_110000;35000;10000_Paldiski_alajaam/LConn2 -- Keila_—_Paldiski_110_kV_CN_35550404_110000_CN_262229346_110000/RConn2
  Keila_—_Paldiski_110_kV_CN_35550404_110000_CN_262229346_110000/RConn3 -- T_35550404_110000;35000;10000_Paldiski_alajaam/LConn3 -- bus84/LConn1
  Järvakandi_—_Valgu_110_kV_CN_35550410_110000_CN_35550412_110000/LConn1 -- T_35550410_110000;10000_Järvakandi_alajaam/LConn1 -- Kehtna_—_Järvakandi_110_kV_CN_35550410_110000_CN_35550415_110000/LConn1
  Järvakandi_—_Valgu_110_kV_CN_35550410_110000_CN_35550412_110000/LConn2 -- T_35550410_110000;10000_Järvakandi_alajaam/LConn2 -- Kehtna_—_Järvakandi_110_kV_CN_35550410_110000_CN_35550415_110000/LConn2
  Järvakandi_—_Valgu_110_kV_CN_35550410_110000_CN_35550412_110000/LConn3 -- T_35550410_110000;10000_Järvakandi_alajaam/LConn3 -- Kehtna_—_Järvakandi_110_kV_CN_35550410_110000_CN_35550415_110000/LConn3 -- bus85/LConn1
  Järvakandi_—_Valgu_110_kV_CN_35550410_110000_CN_35550412_110000/RConn1 -- T_35550412_110000;10000_Valgu_alajaam/LConn1 -- Valgu_—_Vigala_110_kV_CN_35550412_110000_CN_262755193_110000/LConn1
  Järvakandi_—_Valgu_110_kV_CN_35550410_110000_CN_35550412_110000/RConn2 -- T_35550412_110000;10000_Valgu_alajaam/LConn2 -- Valgu_—_Vigala_110_kV_CN_35550412_110000_CN_262755193_110000/LConn2
  Järvakandi_—_Valgu_110_kV_CN_35550410_110000_CN_35550412_110000/RConn3 -- T_35550412_110000;10000_Valgu_alajaam/LConn3 -- Valgu_—_Vigala_110_kV_CN_35550412_110000_CN_262755193_110000/LConn3 -- bus86/LConn1
  T_35550415_110000;10000_Kehtna_alajaam/LConn1 -- Kehtna_—_Järvakandi_110_kV_CN_35550410_110000_CN_35550415_110000/RConn1
  T_35550415_110000;10000_Kehtna_alajaam/LConn2 -- Kehtna_—_Järvakandi_110_kV_CN_35550410_110000_CN_35550415_110000/RConn2
  Kehtna_—_Järvakandi_110_kV_CN_35550410_110000_CN_35550415_110000/RConn3 -- T_35550415_110000;10000_Kehtna_alajaam/LConn3 -- bus87/LConn1
  G_34682060_Balti_Elektrijaam/RConn1 -- _CN_34682059_110000_CN_34682060_110000/RConn1
  G_34682060_Balti_Elektrijaam/RConn2 -- _CN_34682059_110000_CN_34682060_110000/RConn2
  _CN_34682059_110000_CN_34682060_110000/RConn3 -- G_34682060_Balti_Elektrijaam/RConn3 -- bus88/LConn1
  T_321829090_110000;10000_Joala_alajaam/LConn1 -- Balti_EJ_—_Narva_HEJ_110_kV_CN_34682059_110000_CN_321829090_110000/RConn1
  T_321829090_110000;10000_Joala_alajaam/LConn2 -- Balti_EJ_—_Narva_HEJ_110_kV_CN_34682059_110000_CN_321829090_110000/RConn2
  Balti_EJ_—_Narva_HEJ_110_kV_CN_34682059_110000_CN_321829090_110000/RConn3 -- T_321829090_110000;10000_Joala_alajaam/LConn3 -- bus89/LConn1
  T_94121285_110000_Kreenholmi_alajaam/LConn1 -- _CN_34682059_110000_CN_94121285_110000/RConn1
  T_94121285_110000_Kreenholmi_alajaam/LConn2 -- _CN_34682059_110000_CN_94121285_110000/RConn2
  _CN_34682059_110000_CN_94121285_110000/RConn3 -- T_94121285_110000_Kreenholmi_alajaam/LConn3 -- bus90/LConn1
  T_35594708_110000;35000;6000_Narva_Peaalajaam/LConn1 -- _CN_34682059_110000_CN_35594708_110000/RConn1
  T_35594708_110000;35000;6000_Narva_Peaalajaam/LConn2 -- _CN_34682059_110000_CN_35594708_110000/RConn2
  _CN_34682059_110000_CN_35594708_110000/RConn3 -- T_35594708_110000;35000;6000_Narva_Peaalajaam/LConn3 -- bus91/LConn1
  Valgu_—_Vigala_110_kV_CN_35550412_110000_CN_262755193_110000/RConn1 -- T_262755193_110000;10000_Vigala_alajaam/LConn1 -- Lihula_—_Vigala_110_kV_CN_262755193_110000_CN_34988525_110000/LConn1 -- Lihula_—_Vigala_110_kV_CN_262755193_110000_CN_35594731_110000/LConn1 -- Lihula_—_Vigala_110_kV_CN_262755193_110000_CN_34988502_110000/RConn1
  Valgu_—_Vigala_110_kV_CN_35550412_110000_CN_262755193_110000/RConn2 -- T_262755193_110000;10000_Vigala_alajaam/LConn2 -- Lihula_—_Vigala_110_kV_CN_262755193_110000_CN_34988525_110000/LConn2 -- Lihula_—_Vigala_110_kV_CN_262755193_110000_CN_35594731_110000/LConn2 -- Lihula_—_Vigala_110_kV_CN_262755193_110000_CN_34988502_110000/RConn2
  Valgu_—_Vigala_110_kV_CN_35550412_110000_CN_262755193_110000/RConn3 -- T_262755193_110000;10000_Vigala_alajaam/LConn3 -- Lihula_—_Vigala_110_kV_CN_262755193_110000_CN_34988525_110000/LConn3 -- Lihula_—_Vigala_110_kV_CN_262755193_110000_CN_35594731_110000/LConn3 -- Lihula_—_Vigala_110_kV_CN_262755193_110000_CN_34988502_110000/RConn3 -- bus92/LConn1
  T_34968270_110000;10000_Ida_alajaam/LConn1 -- _CN_34968269_110000_CN_34968270_110000/RConn1
  T_34968270_110000;10000_Ida_alajaam/LConn2 -- _CN_34968269_110000_CN_34968270_110000/RConn2
  _CN_34968269_110000_CN_34968270_110000/RConn3 -- T_34968270_110000;10000_Ida_alajaam/LConn3 -- bus93/LConn1
  T_34968274_110000;10000_Viimsi_alajaam/LConn1 -- Kallavere_—_Viimsi_110_kV_CN_34968274_110000_CN_29979106_110000/LConn1
  T_34968274_110000;10000_Viimsi_alajaam/LConn2 -- Kallavere_—_Viimsi_110_kV_CN_34968274_110000_CN_29979106_110000/LConn2
  Kallavere_—_Viimsi_110_kV_CN_34968274_110000_CN_29979106_110000/LConn3 -- T_34968274_110000;10000_Viimsi_alajaam/LConn3 -- bus94/LConn1
  Kallavere_—_Viimsi_110_kV_CN_34968274_110000_CN_29979106_110000/RConn1 -- T_29979106_110000;35000;10000_Kallavere_alajaam/LConn1 -- Iru_—_Kallavere_110_kV_CN_72668114_110000_CN_29979106_110000/RConn1 -- Jägala_haruliin_CN_29978896_110000_CN_29979106_110000/LConn1 -- Aruküla_—_Kallavere_110_kV_CN_204914596_110000_CN_29979106_110000/RConn1 -- _CN_34968276_110000_CN_29979106_110000/LConn1
  Kallavere_—_Viimsi_110_kV_CN_34968274_110000_CN_29979106_110000/RConn2 -- T_29979106_110000;35000;10000_Kallavere_alajaam/LConn2 -- Iru_—_Kallavere_110_kV_CN_72668114_110000_CN_29979106_110000/RConn2 -- Jägala_haruliin_CN_29978896_110000_CN_29979106_110000/LConn2 -- Aruküla_—_Kallavere_110_kV_CN_204914596_110000_CN_29979106_110000/RConn2 -- _CN_34968276_110000_CN_29979106_110000/LConn2
  Kallavere_—_Viimsi_110_kV_CN_34968274_110000_CN_29979106_110000/RConn3 -- T_29979106_110000;35000;10000_Kallavere_alajaam/LConn3 -- Iru_—_Kallavere_110_kV_CN_72668114_110000_CN_29979106_110000/RConn3 -- bus95/LConn1 -- Jägala_haruliin_CN_29978896_110000_CN_29979106_110000/LConn3 -- Aruküla_—_Kallavere_110_kV_CN_204914596_110000_CN_29979106_110000/RConn3 -- _CN_34968276_110000_CN_29979106_110000/LConn3
  T_34968276_110000_Sadama_alajaam/LConn1 -- _CN_34968276_110000_CN_29979106_110000/RConn1
  T_34968276_110000_Sadama_alajaam/LConn2 -- _CN_34968276_110000_CN_29979106_110000/RConn2
  _CN_34968276_110000_CN_29979106_110000/RConn3 -- T_34968276_110000_Sadama_alajaam/LConn3 -- bus96/LConn1
  Voldi_haruliin_CN_101153487_110000_CN_34682089_110000/RConn1 -- T_101153487_110000;15000_Voldi_alajaam/LConn1 -- Voldi_haruliin_CN_101153487_110000_CN_263043288_110000/RConn1 -- Voldi_haruliin_CN_101153487_110000_CN_35594741_110000/LConn1
  Voldi_haruliin_CN_101153487_110000_CN_34682089_110000/RConn2 -- T_101153487_110000;15000_Voldi_alajaam/LConn2 -- Voldi_haruliin_CN_101153487_110000_CN_263043288_110000/RConn2 -- Voldi_haruliin_CN_101153487_110000_CN_35594741_110000/LConn2
  Voldi_haruliin_CN_101153487_110000_CN_34682089_110000/RConn3 -- T_101153487_110000;15000_Voldi_alajaam/LConn3 -- Voldi_haruliin_CN_101153487_110000_CN_263043288_110000/RConn3 -- bus97/LConn1 -- Voldi_haruliin_CN_101153487_110000_CN_35594741_110000/LConn3
  T_35594741_110000;15000;6000;400_Puhja_alajaam/LConn1 -- Voldi_haruliin_CN_101153487_110000_CN_35594741_110000/RConn1
  T_35594741_110000;15000;6000;400_Puhja_alajaam/LConn2 -- Voldi_haruliin_CN_101153487_110000_CN_35594741_110000/RConn2
  Voldi_haruliin_CN_101153487_110000_CN_35594741_110000/RConn3 -- T_35594741_110000;15000;6000;400_Puhja_alajaam/LConn3 -- bus98/LConn1
  T_35555176__/LConn1 -- _CN_34920675_110000_CN_35555176_110000/RConn1
  T_35555176__/LConn2 -- _CN_34920675_110000_CN_35555176_110000/RConn2
  _CN_34920675_110000_CN_35555176_110000/RConn3 -- T_35555176__/LConn3 -- bus99/LConn1
  Püssi_—_Aseri_110_kV_CN_34920675_110000_CN_34920683_110000/RConn1 -- T_34920683_110000;10000_Aseri_alajaam/LConn1 -- Viru_Nigula_—_Aseri_110_kV_CN_34920683_110000_CN_35555175_110000/LConn1 -- Viru_Nigula_—_Aseri_110_kV_CN_34920683_110000_CN_35555173_110000/LConn1
  Püssi_—_Aseri_110_kV_CN_34920675_110000_CN_34920683_110000/RConn2 -- T_34920683_110000;10000_Aseri_alajaam/LConn2 -- Viru_Nigula_—_Aseri_110_kV_CN_34920683_110000_CN_35555175_110000/LConn2 -- Viru_Nigula_—_Aseri_110_kV_CN_34920683_110000_CN_35555173_110000/LConn2
  Püssi_—_Aseri_110_kV_CN_34920675_110000_CN_34920683_110000/RConn3 -- T_34920683_110000;10000_Aseri_alajaam/LConn3 -- Viru_Nigula_—_Aseri_110_kV_CN_34920683_110000_CN_35555175_110000/LConn3 -- Viru_Nigula_—_Aseri_110_kV_CN_34920683_110000_CN_35555173_110000/LConn3 -- bus100/LConn1
  _CN_34903268_110000_CN_35343350_110000/LConn1 -- T_34903268_110000;15000_Imavere_alajaam/LConn1 -- _CN_34903268_110000_CN_34882447_110000/LConn1 -- _CN_34903268_110000_CN_35343349_110000/LConn1 -- _CN_34903268_110000_CN_35343343_110000/RConn1 -- _CN_34903268_110000_CN_35343353_110000/LConn1
  _CN_34903268_110000_CN_35343350_110000/LConn2 -- T_34903268_110000;15000_Imavere_alajaam/LConn2 -- _CN_34903268_110000_CN_34882447_110000/LConn2 -- _CN_34903268_110000_CN_35343349_110000/LConn2 -- _CN_34903268_110000_CN_35343343_110000/RConn2 -- _CN_34903268_110000_CN_35343353_110000/LConn2
  _CN_34903268_110000_CN_35343350_110000/LConn3 -- T_34903268_110000;15000_Imavere_alajaam/LConn3 -- _CN_34903268_110000_CN_34882447_110000/LConn3 -- bus101/LConn1 -- _CN_34903268_110000_CN_35343349_110000/LConn3 -- _CN_34903268_110000_CN_35343343_110000/RConn3 -- _CN_34903268_110000_CN_35343353_110000/LConn3
  T_35343350_110000;35000;10000_Aravete_alajaam/LConn1 -- _CN_34903268_110000_CN_35343350_110000/RConn1
  T_35343350_110000;35000;10000_Aravete_alajaam/LConn2 -- _CN_34903268_110000_CN_35343350_110000/RConn2
  _CN_34903268_110000_CN_35343350_110000/RConn3 -- T_35343350_110000;35000;10000_Aravete_alajaam/LConn3 -- bus102/LConn1
  T_35343349__Roosna_Alliku_alajaam/LConn1 -- _CN_34903268_110000_CN_35343349_110000/RConn1
  T_35343349__Roosna_Alliku_alajaam/LConn2 -- _CN_34903268_110000_CN_35343349_110000/RConn2
  _CN_34903268_110000_CN_35343349_110000/RConn3 -- T_35343349__Roosna_Alliku_alajaam/LConn3 -- bus103/LConn1
  T_35343353_110000;10000_Koigi_alajaam/LConn1 -- _CN_34903268_110000_CN_35343353_110000/RConn1
  T_35343353_110000;10000_Koigi_alajaam/LConn2 -- _CN_34903268_110000_CN_35343353_110000/RConn2
  _CN_34903268_110000_CN_35343353_110000/RConn3 -- T_35343353_110000;10000_Koigi_alajaam/LConn3 -- bus104/LConn1
  _CN_34903268_110000_CN_34882447_110000/RConn1 -- T_34882447_110000;35000;15000;10000_Põltsamaa_alajaam/LConn1 -- Põdra_—_Põltsamaa_110_kV_CN_263282458_110000_CN_34882447_110000/LConn1
  _CN_34903268_110000_CN_34882447_110000/RConn2 -- T_34882447_110000;35000;15000;10000_Põltsamaa_alajaam/LConn2 -- Põdra_—_Põltsamaa_110_kV_CN_263282458_110000_CN_34882447_110000/LConn2
  _CN_34903268_110000_CN_34882447_110000/RConn3 -- T_34882447_110000;35000;15000;10000_Põltsamaa_alajaam/LConn3 -- Põdra_—_Põltsamaa_110_kV_CN_263282458_110000_CN_34882447_110000/LConn3 -- bus105/LConn1
  T_30222062_110000;10000_Emajõe_alajaam/LConn1 -- Tartu_—_Emajõe_110_kV_CN_34682089_110000_CN_30222062_110000/RConn1
  T_30222062_110000;10000_Emajõe_alajaam/LConn2 -- Tartu_—_Emajõe_110_kV_CN_34682089_110000_CN_30222062_110000/RConn2
  Tartu_—_Emajõe_110_kV_CN_34682089_110000_CN_30222062_110000/RConn3 -- T_30222062_110000;10000_Emajõe_alajaam/LConn3 -- bus106/LConn1
  Viru_Nigula_—_Aseri_110_kV_CN_34920683_110000_CN_35555175_110000/RConn1 -- T_35555175_110000;20000;10000;6000_Kunda_alajaam/LConn1 -- Haljala_haruliin_CN_34920691_110000_CN_35555175_110000/LConn1
  Viru_Nigula_—_Aseri_110_kV_CN_34920683_110000_CN_35555175_110000/RConn2 -- T_35555175_110000;20000;10000;6000_Kunda_alajaam/LConn2 -- Haljala_haruliin_CN_34920691_110000_CN_35555175_110000/LConn2
  Viru_Nigula_—_Aseri_110_kV_CN_34920683_110000_CN_35555175_110000/RConn3 -- T_35555175_110000;20000;10000;6000_Kunda_alajaam/LConn3 -- Haljala_haruliin_CN_34920691_110000_CN_35555175_110000/LConn3 -- bus107/LConn1
  T_35555173_110000_Viru_Nigula_alajaam/LConn1 -- Viru_Nigula_—_Aseri_110_kV_CN_34920683_110000_CN_35555173_110000/RConn1
  T_35555173_110000_Viru_Nigula_alajaam/LConn2 -- Viru_Nigula_—_Aseri_110_kV_CN_34920683_110000_CN_35555173_110000/RConn2
  Viru_Nigula_—_Aseri_110_kV_CN_34920683_110000_CN_35555173_110000/RConn3 -- T_35555173_110000_Viru_Nigula_alajaam/LConn3 -- bus108/LConn1
  Haljala_haruliin_CN_34920691_110000_CN_34920699_110000/RConn1 -- T_34920691_110000;35000;10000_Haljala_alajaam/LConn1 -- Haljala_haruliin_CN_34920691_110000_CN_35555175_110000/RConn1 -- Haljala_haruliin_CN_34920691_110000_CN_35555163_110000/LConn1 -- Haljala_haruliin_CN_34920691_110000_CN_35555166_110000/LConn1 -- Haljala_haruliin_CN_34920691_110000_CN_35555165_110000/LConn1 -- Haljala_haruliin_CN_34920691_110000_CN_35555161_110000/LConn1
  Haljala_haruliin_CN_34920691_110000_CN_34920699_110000/RConn2 -- T_34920691_110000;35000;10000_Haljala_alajaam/LConn2 -- Haljala_haruliin_CN_34920691_110000_CN_35555175_110000/RConn2 -- Haljala_haruliin_CN_34920691_110000_CN_35555163_110000/LConn2 -- Haljala_haruliin_CN_34920691_110000_CN_35555166_110000/LConn2 -- Haljala_haruliin_CN_34920691_110000_CN_35555165_110000/LConn2 -- Haljala_haruliin_CN_34920691_110000_CN_35555161_110000/LConn2
  Haljala_haruliin_CN_34920691_110000_CN_34920699_110000/RConn3 -- T_34920691_110000;35000;10000_Haljala_alajaam/LConn3 -- Haljala_haruliin_CN_34920691_110000_CN_35555175_110000/RConn3 -- bus109/LConn1 -- Haljala_haruliin_CN_34920691_110000_CN_35555163_110000/LConn3 -- Haljala_haruliin_CN_34920691_110000_CN_35555166_110000/LConn3 -- Haljala_haruliin_CN_34920691_110000_CN_35555165_110000/LConn3 -- Haljala_haruliin_CN_34920691_110000_CN_35555161_110000/LConn3
  T_35555163_110000;10000_Viitna_alajaam/LConn1 -- Haljala_haruliin_CN_34920691_110000_CN_35555163_110000/RConn1
  T_35555163_110000;10000_Viitna_alajaam/LConn2 -- Haljala_haruliin_CN_34920691_110000_CN_35555163_110000/RConn2
  Haljala_haruliin_CN_34920691_110000_CN_35555163_110000/RConn3 -- T_35555163_110000;10000_Viitna_alajaam/LConn3 -- bus110/LConn1
  Haljala_haruliin_CN_34920691_110000_CN_35555166_110000/RConn1 -- T_35555166_110000;10000_Loksa_alajaam/LConn1 -- Kuusalu_—_Kolga_110_kV_CN_35384083_110000_CN_35555166_110000/LConn1
  Haljala_haruliin_CN_34920691_110000_CN_35555166_110000/RConn2 -- T_35555166_110000;10000_Loksa_alajaam/LConn2 -- Kuusalu_—_Kolga_110_kV_CN_35384083_110000_CN_35555166_110000/LConn2
  Haljala_haruliin_CN_34920691_110000_CN_35555166_110000/RConn3 -- T_35555166_110000;10000_Loksa_alajaam/LConn3 -- Kuusalu_—_Kolga_110_kV_CN_35384083_110000_CN_35555166_110000/LConn3 -- bus111/LConn1
  T_35555165_110000;10000_Võsu_alajaam/LConn1 -- Haljala_haruliin_CN_34920691_110000_CN_35555165_110000/RConn1
  T_35555165_110000;10000_Võsu_alajaam/LConn2 -- Haljala_haruliin_CN_34920691_110000_CN_35555165_110000/RConn2
  Haljala_haruliin_CN_34920691_110000_CN_35555165_110000/RConn3 -- T_35555165_110000;10000_Võsu_alajaam/LConn3 -- bus112/LConn1
  T_35555161_110000;10000_Kadrina_alajaam/LConn1 -- Haljala_haruliin_CN_34920691_110000_CN_35555161_110000/RConn1
  T_35555161_110000;10000_Kadrina_alajaam/LConn2 -- Haljala_haruliin_CN_34920691_110000_CN_35555161_110000/RConn2
  Haljala_haruliin_CN_34920691_110000_CN_35555161_110000/RConn3 -- T_35555161_110000;10000_Kadrina_alajaam/LConn3 -- bus113/LConn1
  T_36977398_110000;15000_Oiu_alajaam/LConn1 -- Oiu_haruliin_CN_36977398_110000_CN_180118919_110000/LConn1
  T_36977398_110000;15000_Oiu_alajaam/LConn2 -- Oiu_haruliin_CN_36977398_110000_CN_180118919_110000/LConn2
  Oiu_haruliin_CN_36977398_110000_CN_180118919_110000/LConn3 -- T_36977398_110000;15000_Oiu_alajaam/LConn3 -- bus114/LConn1
  Oiu_haruliin_CN_36977398_110000_CN_180118919_110000/RConn1 -- T_180118919_110000;15000;10000_Saare_alajaam/LConn1 -- Saare_—_Mustvee_110_kV_CN_35451776_110000_CN_180118919_110000/RConn1
  Oiu_haruliin_CN_36977398_110000_CN_180118919_110000/RConn2 -- T_180118919_110000;15000;10000_Saare_alajaam/LConn2 -- Saare_—_Mustvee_110_kV_CN_35451776_110000_CN_180118919_110000/RConn2
  Oiu_haruliin_CN_36977398_110000_CN_180118919_110000/RConn3 -- T_180118919_110000;15000;10000_Saare_alajaam/LConn3 -- Saare_—_Mustvee_110_kV_CN_35451776_110000_CN_180118919_110000/RConn3 -- bus115/LConn1
  T_263253461_110000;10000_Ruusmäe_alajaam/LConn1 -- _CN_263253461_110000_CN_182242759_110000/RConn1
  T_263253461_110000;10000_Ruusmäe_alajaam/LConn2 -- _CN_263253461_110000_CN_182242759_110000/RConn2
  _CN_263253461_110000_CN_182242759_110000/RConn3 -- T_263253461_110000;10000_Ruusmäe_alajaam/LConn3 -- bus116/LConn1
  Muhu_haruliin_CN_35022081_110000_CN_34988518_110000/LConn1 -- T_35022081_110000;10000_Muhu_alajaam/LConn1 -- Muhu_haruliin_CN_35022081_110000_CN_34988522_110000/LConn1
  Muhu_haruliin_CN_35022081_110000_CN_34988518_110000/LConn2 -- T_35022081_110000;10000_Muhu_alajaam/LConn2 -- Muhu_haruliin_CN_35022081_110000_CN_34988522_110000/LConn2
  Muhu_haruliin_CN_35022081_110000_CN_34988518_110000/LConn3 -- T_35022081_110000;10000_Muhu_alajaam/LConn3 -- Muhu_haruliin_CN_35022081_110000_CN_34988522_110000/LConn3 -- bus117/LConn1
  T_34988518_110000;35000;10000_Võiküla_alajaam/LConn1 -- Muhu_haruliin_CN_35022081_110000_CN_34988518_110000/RConn1
  T_34988518_110000;35000;10000_Võiküla_alajaam/LConn2 -- Muhu_haruliin_CN_35022081_110000_CN_34988518_110000/RConn2
  Muhu_haruliin_CN_35022081_110000_CN_34988518_110000/RConn3 -- T_34988518_110000;35000;10000_Võiküla_alajaam/LConn3 -- bus118/LConn1
  T_34988522_110000;35000;10000_Tusti_alajaam/LConn1 -- Muhu_haruliin_CN_35022081_110000_CN_34988522_110000/RConn1
  T_34988522_110000;35000;10000_Tusti_alajaam/LConn2 -- Muhu_haruliin_CN_35022081_110000_CN_34988522_110000/RConn2
  Muhu_haruliin_CN_35022081_110000_CN_34988522_110000/RConn3 -- T_34988522_110000;35000;10000_Tusti_alajaam/LConn3 -- bus119/LConn1
  T_29978896_110000;20000_Jägala_alajaam/LConn1 -- Jägala_haruliin_CN_29978896_110000_CN_29979106_110000/RConn1
  T_29978896_110000;20000_Jägala_alajaam/LConn2 -- Jägala_haruliin_CN_29978896_110000_CN_29979106_110000/RConn2
  Jägala_haruliin_CN_29978896_110000_CN_29979106_110000/RConn3 -- T_29978896_110000;20000_Jägala_alajaam/LConn3 -- bus120/LConn1
  Kuusalu_—_Kolga_110_kV_CN_35384083_110000_CN_35555166_110000/RConn1 -- T_35384083_110000;35000;10000_Kuusalu_alajaam/LConn1 -- Kuusalu_—_Kolga_110_kV_CN_35384083_110000_CN_35555171_110000/LConn1
  Kuusalu_—_Kolga_110_kV_CN_35384083_110000_CN_35555166_110000/RConn2 -- T_35384083_110000;35000;10000_Kuusalu_alajaam/LConn2 -- Kuusalu_—_Kolga_110_kV_CN_35384083_110000_CN_35555171_110000/LConn2
  Kuusalu_—_Kolga_110_kV_CN_35384083_110000_CN_35555166_110000/RConn3 -- T_35384083_110000;35000;10000_Kuusalu_alajaam/LConn3 -- Kuusalu_—_Kolga_110_kV_CN_35384083_110000_CN_35555171_110000/LConn3 -- bus121/LConn1
  T_35555171_110000;10000_Kolga_alajaam/LConn1 -- Kuusalu_—_Kolga_110_kV_CN_35384083_110000_CN_35555171_110000/RConn1
  T_35555171_110000;10000_Kolga_alajaam/LConn2 -- Kuusalu_—_Kolga_110_kV_CN_35384083_110000_CN_35555171_110000/RConn2
  Kuusalu_—_Kolga_110_kV_CN_35384083_110000_CN_35555171_110000/RConn3 -- T_35555171_110000;10000_Kolga_alajaam/LConn3 -- bus122/LConn1
  Jõgeva_—_Põdra_110_kV_CN_263282458_110000_CN_35451774_110000/RConn1 -- T_263282458_110000;10000_Põdra_alajaam/LConn1 -- Põdra_—_Põltsamaa_110_kV_CN_263282458_110000_CN_34882447_110000/RConn1
  Jõgeva_—_Põdra_110_kV_CN_263282458_110000_CN_35451774_110000/RConn2 -- T_263282458_110000;10000_Põdra_alajaam/LConn2 -- Põdra_—_Põltsamaa_110_kV_CN_263282458_110000_CN_34882447_110000/RConn2
  Jõgeva_—_Põdra_110_kV_CN_263282458_110000_CN_35451774_110000/RConn3 -- T_263282458_110000;10000_Põdra_alajaam/LConn3 -- Põdra_—_Põltsamaa_110_kV_CN_263282458_110000_CN_34882447_110000/RConn3 -- bus123/LConn1
  Keila_—_Rummu_110_kV_CN_262229346_110000_CN_34988486_110000/RConn1 -- T_34988486_110000;35000;10000_Rummu_alajaam/LConn1 -- Rummu_—_Nõva_110_kV_CN_34988486_110000_CN_34988495_110000/LConn1
  Keila_—_Rummu_110_kV_CN_262229346_110000_CN_34988486_110000/RConn2 -- T_34988486_110000;35000;10000_Rummu_alajaam/LConn2 -- Rummu_—_Nõva_110_kV_CN_34988486_110000_CN_34988495_110000/LConn2
  Keila_—_Rummu_110_kV_CN_262229346_110000_CN_34988486_110000/RConn3 -- T_34988486_110000;35000;10000_Rummu_alajaam/LConn3 -- Rummu_—_Nõva_110_kV_CN_34988486_110000_CN_34988495_110000/LConn3 -- bus124/LConn1
  Lihula_—_Vigala_110_kV_CN_262755193_110000_CN_34988525_110000/RConn1 -- T_34988525_110000;10000_Martna_alajaam/LConn1 -- Aulepa_—_Taebla_110_kV_CN_101177924_110000_CN_34988525_110000/LConn1
  Lihula_—_Vigala_110_kV_CN_262755193_110000_CN_34988525_110000/RConn2 -- T_34988525_110000;10000_Martna_alajaam/LConn2 -- Aulepa_—_Taebla_110_kV_CN_101177924_110000_CN_34988525_110000/LConn2
  Lihula_—_Vigala_110_kV_CN_262755193_110000_CN_34988525_110000/RConn3 -- T_34988525_110000;10000_Martna_alajaam/LConn3 -- Aulepa_—_Taebla_110_kV_CN_101177924_110000_CN_34988525_110000/LConn3 -- bus125/LConn1
  T_35594731_110000;10000_Kullamaa_alajaam/LConn1 -- Lihula_—_Vigala_110_kV_CN_262755193_110000_CN_35594731_110000/RConn1
  T_35594731_110000;10000_Kullamaa_alajaam/LConn2 -- Lihula_—_Vigala_110_kV_CN_262755193_110000_CN_35594731_110000/RConn2
  Lihula_—_Vigala_110_kV_CN_262755193_110000_CN_35594731_110000/RConn3 -- T_35594731_110000;10000_Kullamaa_alajaam/LConn3 -- bus126/LConn1
  Aulepa_—_Taebla_110_kV_CN_101177924_110000_CN_34988531_110000/LConn1 -- T_101177924_110000_Aulepa_alajaam/LConn1 -- Aulepa_—_Taebla_110_kV_CN_101177924_110000_CN_34988527_110000/LConn1 -- Aulepa_—_Taebla_110_kV_CN_101177924_110000_CN_34988525_110000/RConn1 -- Nõva_—_Aulepa_110_kV_CN_101177924_110000_CN_34988495_110000/LConn1
  Aulepa_—_Taebla_110_kV_CN_101177924_110000_CN_34988531_110000/LConn2 -- T_101177924_110000_Aulepa_alajaam/LConn2 -- Aulepa_—_Taebla_110_kV_CN_101177924_110000_CN_34988527_110000/LConn2 -- Aulepa_—_Taebla_110_kV_CN_101177924_110000_CN_34988525_110000/RConn2 -- Nõva_—_Aulepa_110_kV_CN_101177924_110000_CN_34988495_110000/LConn2
  Aulepa_—_Taebla_110_kV_CN_101177924_110000_CN_34988531_110000/LConn3 -- T_101177924_110000_Aulepa_alajaam/LConn3 -- Aulepa_—_Taebla_110_kV_CN_101177924_110000_CN_34988527_110000/LConn3 -- Aulepa_—_Taebla_110_kV_CN_101177924_110000_CN_34988525_110000/RConn3 -- Nõva_—_Aulepa_110_kV_CN_101177924_110000_CN_34988495_110000/LConn3 -- bus127/LConn1
  T_34988531_110000;10000_Taebla_alajaam/LConn1 -- Aulepa_—_Taebla_110_kV_CN_101177924_110000_CN_34988531_110000/RConn1
  T_34988531_110000;10000_Taebla_alajaam/LConn2 -- Aulepa_—_Taebla_110_kV_CN_101177924_110000_CN_34988531_110000/RConn2
  Aulepa_—_Taebla_110_kV_CN_101177924_110000_CN_34988531_110000/RConn3 -- T_34988531_110000;10000_Taebla_alajaam/LConn3 -- bus128/LConn1
  T_34988527_110000;35000;10000_Haapsalu_alajaam/LConn1 -- Aulepa_—_Taebla_110_kV_CN_101177924_110000_CN_34988527_110000/RConn1
  T_34988527_110000;35000;10000_Haapsalu_alajaam/LConn2 -- Aulepa_—_Taebla_110_kV_CN_101177924_110000_CN_34988527_110000/RConn2
  Aulepa_—_Taebla_110_kV_CN_101177924_110000_CN_34988527_110000/RConn3 -- T_34988527_110000;35000;10000_Haapsalu_alajaam/LConn3 -- bus129/LConn1
  Nõva_—_Aulepa_110_kV_CN_101177924_110000_CN_34988495_110000/RConn1 -- T_34988495_110000;10000_Nõva_alajaam/LConn1 -- Rummu_—_Nõva_110_kV_CN_34988486_110000_CN_34988495_110000/RConn1
  Nõva_—_Aulepa_110_kV_CN_101177924_110000_CN_34988495_110000/RConn2 -- T_34988495_110000;10000_Nõva_alajaam/LConn2 -- Rummu_—_Nõva_110_kV_CN_34988486_110000_CN_34988495_110000/RConn2
  Nõva_—_Aulepa_110_kV_CN_101177924_110000_CN_34988495_110000/RConn3 -- T_34988495_110000;10000_Nõva_alajaam/LConn3 -- Rummu_—_Nõva_110_kV_CN_34988486_110000_CN_34988495_110000/RConn3 -- bus130/LConn1
  Harku_—_Aruküla_330_kV_CN_34968224_330000_CN_34935436_330000/LConn1 -- T_34968224_330000;110000;20000_Harku_ajajaam/LConn1 -- Harku_—_Aruküla_330_kV_CN_34968224_330000_CN_204914596_330000/LConn1 -- Harku_—_Aruküla_330_kV_CN_34968224_330000_CN_34682059_330000/LConn1
  Harku_—_Aruküla_330_kV_CN_34968224_330000_CN_34935436_330000/LConn2 -- T_34968224_330000;110000;20000_Harku_ajajaam/LConn2 -- Harku_—_Aruküla_330_kV_CN_34968224_330000_CN_204914596_330000/LConn2 -- Harku_—_Aruküla_330_kV_CN_34968224_330000_CN_34682059_330000/LConn2
  Harku_—_Aruküla_330_kV_CN_34968224_330000_CN_34935436_330000/LConn3 -- T_34968224_330000;110000;20000_Harku_ajajaam/LConn3 -- Harku_—_Aruküla_330_kV_CN_34968224_330000_CN_204914596_330000/LConn3 -- Harku_—_Aruküla_330_kV_CN_34968224_330000_CN_34682059_330000/LConn3 -- bus131/LConn1
  Harku_—_Aruküla_330_kV_CN_34968224_330000_CN_34935436_330000/RConn1 -- T_34935436_330000;220000;110000;35000;10000_Kiisa_alajaam/LConn1 -- Püssi_—_Rakvere_330_kV_CN_34920675_330000_CN_34935436_330000/LConn1 -- _CN_34935436_330000_CN_265791084_110000/RConn1 -- Paide_—_Kiisa_330_kV_CN_34935436_330000_CN_35343343_330000/LConn1
  Harku_—_Aruküla_330_kV_CN_34968224_330000_CN_34935436_330000/RConn2 -- T_34935436_330000;220000;110000;35000;10000_Kiisa_alajaam/LConn2 -- Püssi_—_Rakvere_330_kV_CN_34920675_330000_CN_34935436_330000/LConn2 -- _CN_34935436_330000_CN_265791084_110000/RConn2 -- Paide_—_Kiisa_330_kV_CN_34935436_330000_CN_35343343_330000/LConn2
  Harku_—_Aruküla_330_kV_CN_34968224_330000_CN_34935436_330000/RConn3 -- T_34935436_330000;220000;110000;35000;10000_Kiisa_alajaam/LConn3 -- Püssi_—_Rakvere_330_kV_CN_34920675_330000_CN_34935436_330000/LConn3 -- _CN_34935436_330000_CN_265791084_110000/RConn3 -- Paide_—_Kiisa_330_kV_CN_34935436_330000_CN_35343343_330000/LConn3 -- bus132/LConn1
  T_204914596_330000;110000;10000_Aruküla_330kV_alajaam/LConn1 -- Harku_—_Aruküla_330_kV_CN_34968224_330000_CN_204914596_330000/RConn1
  T_204914596_330000;110000;10000_Aruküla_330kV_alajaam/LConn2 -- Harku_—_Aruküla_330_kV_CN_34968224_330000_CN_204914596_330000/RConn2
  Harku_—_Aruküla_330_kV_CN_34968224_330000_CN_204914596_330000/RConn3 -- T_204914596_330000;110000;10000_Aruküla_330kV_alajaam/LConn3 -- bus133/LConn1
  Harku_—_Aruküla_330_kV_CN_34968224_330000_CN_34682059_330000/RConn1 -- T_34682059_330000;110000_Balti_EJ_alajaam/LConn1 -- Balti_EJ_—_Püssi_330_kV_CN_34920675_330000_CN_34682059_330000/LConn1 -- Balti_—_Tartu_330_kV_&_Tartu_—_Viljandi_330_kV_CN_34682089_330000_CN_34682059_330000/LConn1 -- _CN_34682059_330000_CN_34682061_330000/LConn1 -- Eesti_EJ_—_Balti_EJ_330_kV_CN_34682059_330000_CN_34685101_330000/LConn1
  Harku_—_Aruküla_330_kV_CN_34968224_330000_CN_34682059_330000/RConn2 -- T_34682059_330000;110000_Balti_EJ_alajaam/LConn2 -- Balti_EJ_—_Püssi_330_kV_CN_34920675_330000_CN_34682059_330000/LConn2 -- Balti_—_Tartu_330_kV_&_Tartu_—_Viljandi_330_kV_CN_34682089_330000_CN_34682059_330000/LConn2 -- _CN_34682059_330000_CN_34682061_330000/LConn2 -- Eesti_EJ_—_Balti_EJ_330_kV_CN_34682059_330000_CN_34685101_330000/LConn2
  Harku_—_Aruküla_330_kV_CN_34968224_330000_CN_34682059_330000/RConn3 -- T_34682059_330000;110000_Balti_EJ_alajaam/LConn3 -- Balti_EJ_—_Püssi_330_kV_CN_34920675_330000_CN_34682059_330000/LConn3 -- Balti_—_Tartu_330_kV_&_Tartu_—_Viljandi_330_kV_CN_34682089_330000_CN_34682059_330000/LConn3 -- _CN_34682059_330000_CN_34682061_330000/LConn3 -- Eesti_EJ_—_Balti_EJ_330_kV_CN_34682059_330000_CN_34685101_330000/LConn3 -- bus134/LConn1
  Püssi_—_Rakvere_330_kV_CN_34920675_330000_CN_34935436_330000/RConn1 -- T_34920675_330000;220000;110000;10000_Püssi_alajaam/LConn1 -- Eesti_EJ_—_Püssi_330_kV_CN_34920675_330000_CN_34685101_330000/LConn1 -- Balti_EJ_—_Püssi_330_kV_CN_34920675_330000_CN_34682059_330000/RConn1 -- Püssi_—_Rakvere_330_kV_CN_34920675_330000_CN_34920699_330000/LConn1
  Püssi_—_Rakvere_330_kV_CN_34920675_330000_CN_34935436_330000/RConn2 -- T_34920675_330000;220000;110000;10000_Püssi_alajaam/LConn2 -- Eesti_EJ_—_Püssi_330_kV_CN_34920675_330000_CN_34685101_330000/LConn2 -- Balti_EJ_—_Püssi_330_kV_CN_34920675_330000_CN_34682059_330000/RConn2 -- Püssi_—_Rakvere_330_kV_CN_34920675_330000_CN_34920699_330000/LConn2
  Püssi_—_Rakvere_330_kV_CN_34920675_330000_CN_34935436_330000/RConn3 -- T_34920675_330000;220000;110000;10000_Püssi_alajaam/LConn3 -- Eesti_EJ_—_Püssi_330_kV_CN_34920675_330000_CN_34685101_330000/LConn3 -- Balti_EJ_—_Püssi_330_kV_CN_34920675_330000_CN_34682059_330000/RConn3 -- bus135/LConn1 -- Püssi_—_Rakvere_330_kV_CN_34920675_330000_CN_34920699_330000/LConn3
  T_34920699_330000;110000;35000;10000_Rakvere_alajaam/LConn1 -- Püssi_—_Rakvere_330_kV_CN_34920675_330000_CN_34920699_330000/RConn1
  T_34920699_330000;110000;35000;10000_Rakvere_alajaam/LConn2 -- Püssi_—_Rakvere_330_kV_CN_34920675_330000_CN_34920699_330000/RConn2
  Püssi_—_Rakvere_330_kV_CN_34920675_330000_CN_34920699_330000/RConn3 -- T_34920699_330000;110000;35000;10000_Rakvere_alajaam/LConn3 -- bus136/LConn1
  Eesti_EJ_—_Püssi_330_kV_CN_34920675_330000_CN_34685101_330000/RConn1 -- T_34685101_330000_Eesti_EJ_alajaam/LConn1 -- Eesti_EJ_—_Balti_EJ_330_kV_CN_34682059_330000_CN_34685101_330000/RConn1 -- _CN_34685101_330000_CN_34685113_330000/LConn1 -- Eesti_EJ_—_Paide_330_kV_CN_34685101_330000_CN_35343343_330000/LConn1
  Eesti_EJ_—_Püssi_330_kV_CN_34920675_330000_CN_34685101_330000/RConn2 -- T_34685101_330000_Eesti_EJ_alajaam/LConn2 -- Eesti_EJ_—_Balti_EJ_330_kV_CN_34682059_330000_CN_34685101_330000/RConn2 -- _CN_34685101_330000_CN_34685113_330000/LConn2 -- Eesti_EJ_—_Paide_330_kV_CN_34685101_330000_CN_35343343_330000/LConn2
  Eesti_EJ_—_Püssi_330_kV_CN_34920675_330000_CN_34685101_330000/RConn3 -- T_34685101_330000_Eesti_EJ_alajaam/LConn3 -- Eesti_EJ_—_Balti_EJ_330_kV_CN_34682059_330000_CN_34685101_330000/RConn3 -- _CN_34685101_330000_CN_34685113_330000/LConn3 -- Eesti_EJ_—_Paide_330_kV_CN_34685101_330000_CN_35343343_330000/LConn3 -- bus137/LConn1
  Balti_—_Tartu_330_kV_&_Tartu_—_Viljandi_330_kV_CN_34682089_330000_CN_34682059_330000/RConn1 -- T_34682089_330000;110000;35000;15000;10000_Tartu_alajaam/LConn1 -- Balti_—_Tartu_330_kV_&_Tartu_—_Viljandi_330_kV_CN_34682089_330000_CN_35450930_330000/LConn1
  Balti_—_Tartu_330_kV_&_Tartu_—_Viljandi_330_kV_CN_34682089_330000_CN_34682059_330000/RConn2 -- T_34682089_330000;110000;35000;15000;10000_Tartu_alajaam/LConn2 -- Balti_—_Tartu_330_kV_&_Tartu_—_Viljandi_330_kV_CN_34682089_330000_CN_35450930_330000/LConn2
  Balti_—_Tartu_330_kV_&_Tartu_—_Viljandi_330_kV_CN_34682089_330000_CN_34682059_330000/RConn3 -- T_34682089_330000;110000;35000;15000;10000_Tartu_alajaam/LConn3 -- Balti_—_Tartu_330_kV_&_Tartu_—_Viljandi_330_kV_CN_34682089_330000_CN_35450930_330000/LConn3 -- bus138/LConn1
  Balti_—_Tartu_330_kV_&_Tartu_—_Viljandi_330_kV_CN_34682089_330000_CN_35450930_330000/RConn1 -- T_35450930_330000;110000_Sindi_alajaam/LConn1 -- Paide_—_Sindi_330_kV_CN_35343343_330000_CN_35450930_330000/LConn1
  Balti_—_Tartu_330_kV_&_Tartu_—_Viljandi_330_kV_CN_34682089_330000_CN_35450930_330000/RConn2 -- T_35450930_330000;110000_Sindi_alajaam/LConn2 -- Paide_—_Sindi_330_kV_CN_35343343_330000_CN_35450930_330000/LConn2
  Balti_—_Tartu_330_kV_&_Tartu_—_Viljandi_330_kV_CN_34682089_330000_CN_35450930_330000/RConn3 -- T_35450930_330000;110000_Sindi_alajaam/LConn3 -- Paide_—_Sindi_330_kV_CN_35343343_330000_CN_35450930_330000/LConn3 -- bus139/LConn1
  G_34682061_/RConn1 -- _CN_34682059_330000_CN_34682061_330000/RConn1
  G_34682061_/RConn2 -- _CN_34682059_330000_CN_34682061_330000/RConn2
  _CN_34682059_330000_CN_34682061_330000/RConn3 -- G_34682061_/RConn3 -- bus140/LConn1
  Paide_—_Kiisa_330_kV_CN_34935436_330000_CN_35343343_330000/RConn1 -- T_35343343_330000;110000;35000;10000_Paide_alajaam/LConn1 -- Eesti_EJ_—_Paide_330_kV_CN_34685101_330000_CN_35343343_330000/RConn1 -- Paide_—_Sindi_330_kV_CN_35343343_330000_CN_35450930_330000/RConn1
  Paide_—_Kiisa_330_kV_CN_34935436_330000_CN_35343343_330000/RConn2 -- T_35343343_330000;110000;35000;10000_Paide_alajaam/LConn2 -- Eesti_EJ_—_Paide_330_kV_CN_34685101_330000_CN_35343343_330000/RConn2 -- Paide_—_Sindi_330_kV_CN_35343343_330000_CN_35450930_330000/RConn2
  Paide_—_Kiisa_330_kV_CN_34935436_330000_CN_35343343_330000/RConn3 -- T_35343343_330000;110000;35000;10000_Paide_alajaam/LConn3 -- Eesti_EJ_—_Paide_330_kV_CN_34685101_330000_CN_35343343_330000/RConn3 -- Paide_—_Sindi_330_kV_CN_35343343_330000_CN_35450930_330000/RConn3 -- bus141/LConn1
  T_34685113_330000;110000;35000;10000_Tsinguliina_alajaam/LConn1 -- _CN_34685101_330000_CN_34685113_330000/RConn1
  T_34685113_330000;110000;35000;10000_Tsinguliina_alajaam/LConn2 -- _CN_34685101_330000_CN_34685113_330000/RConn2
  _CN_34685101_330000_CN_34685113_330000/RConn3 -- T_34685113_330000;110000;35000;10000_Tsinguliina_alajaam/LConn3 -- bus142/LConn1
  T_35379726_110000;35000;10000_Kehra_alajaam/RConn1 -- L_35379726/LConn1
  T_35379726_110000;35000;10000_Kehra_alajaam/RConn2 -- L_35379726/LConn2
  L_35379726/LConn3 -- T_35379726_110000;35000;10000_Kehra_alajaam/RConn3 -- bus143/LConn1
  T_35384064_110000;35000;10000_Tapa_alajaam/RConn1 -- L_35384064/LConn1
  T_35384064_110000;35000;10000_Tapa_alajaam/RConn2 -- L_35384064/LConn2
  L_35384064/LConn3 -- T_35384064_110000;35000;10000_Tapa_alajaam/RConn3 -- bus144/LConn1
  T_264287766_110000_PTK_alajaam/RConn1 -- L_264287766/LConn1
  T_264287766_110000_PTK_alajaam/RConn2 -- L_264287766/LConn2
  L_264287766/LConn3 -- T_264287766_110000_PTK_alajaam/RConn3 -- bus145/LConn1
  T_139400061_110000;35000;6000_Eesti_EJ_OT_alajaam/RConn1 -- L_139400061/LConn1
  T_139400061_110000;35000;6000_Eesti_EJ_OT_alajaam/RConn2 -- L_139400061/LConn2
  L_139400061/LConn3 -- T_139400061_110000;35000;6000_Eesti_EJ_OT_alajaam/RConn3 -- bus146/LConn1
  T_35367480_110000;35000_Sirgala_alajaam/RConn1 -- L_35367480/LConn1
  T_35367480_110000;35000_Sirgala_alajaam/RConn2 -- L_35367480/LConn2
  L_35367480/LConn3 -- T_35367480_110000;35000_Sirgala_alajaam/RConn3 -- bus147/LConn1
  T_35594697_110000;6000_Pargi_alajaam/RConn1 -- L_35594697/LConn1
  T_35594697_110000;6000_Pargi_alajaam/RConn2 -- L_35594697/LConn2
  L_35594697/LConn3 -- T_35594697_110000;6000_Pargi_alajaam/RConn3 -- bus148/LConn1
  T_205980356_110000;35000;6000_Ahtme_alajaam/RConn1 -- L_205980356/LConn1
  T_205980356_110000;35000;6000_Ahtme_alajaam/RConn2 -- L_205980356/LConn2
  L_205980356/LConn3 -- T_205980356_110000;35000;6000_Ahtme_alajaam/RConn3 -- bus149/LConn1
  T_35450914_110000;35000;10000_Pärnu_Jaagupi_alajaam/RConn1 -- L_35450914/LConn1
  T_35450914_110000;35000;10000_Pärnu_Jaagupi_alajaam/RConn2 -- L_35450914/LConn2
  L_35450914/LConn3 -- T_35450914_110000;35000;10000_Pärnu_Jaagupi_alajaam/RConn3 -- bus150/LConn1
  T_35450940_110000;35000;10000_Vändra_alajaam/RConn1 -- L_35450940/LConn1
  T_35450940_110000;35000;10000_Vändra_alajaam/RConn2 -- L_35450940/LConn2
  L_35450940/LConn3 -- T_35450940_110000;35000;10000_Vändra_alajaam/RConn3 -- bus151/LConn1
  T_35445361_110000;35000;15000_Kilingi_Nõmme_alajaam/RConn1 -- L_35445361/LConn1
  T_35445361_110000;35000;15000_Kilingi_Nõmme_alajaam/RConn2 -- L_35445361/LConn2
  L_35445361/LConn3 -- T_35445361_110000;35000;15000_Kilingi_Nõmme_alajaam/RConn3 -- bus152/LConn1
  T_263043288_110000;35000;15000;6000_Viljandi_alajaam/RConn1 -- L_263043288/LConn1
  T_263043288_110000;35000;15000;6000_Viljandi_alajaam/RConn2 -- L_263043288/LConn2
  L_263043288/LConn3 -- T_263043288_110000;35000;15000;6000_Viljandi_alajaam/RConn3 -- bus153/LConn1
  T_35450875_110000;10000_Kabli_alajaam/RConn1 -- L_35450875/LConn1
  T_35450875_110000;10000_Kabli_alajaam/RConn2 -- L_35450875/LConn2
  L_35450875/LConn3 -- T_35450875_110000;10000_Kabli_alajaam/RConn3 -- bus154/LConn1
  T_263962720_110000;10000_Paikuse_alajaam/RConn1 -- L_263962720/LConn1
  T_263962720_110000;10000_Paikuse_alajaam/RConn2 -- L_263962720/LConn2
  L_263962720/LConn3 -- T_263962720_110000;10000_Paikuse_alajaam/RConn3 -- bus155/LConn1
  T_35450920_110000;10000_Lõpe_alajaam/RConn1 -- L_35450920/LConn1
  T_35450920_110000;10000_Lõpe_alajaam/RConn2 -- L_35450920/LConn2
  L_35450920/LConn3 -- T_35450920_110000;10000_Lõpe_alajaam/RConn3 -- bus156/LConn1
  T_35450919_110000;35000;10000_Audru_alajaam/RConn1 -- L_35450919/LConn1
  T_35450919_110000;35000;10000_Audru_alajaam/RConn2 -- L_35450919/LConn2
  L_35450919/LConn3 -- T_35450919_110000;35000;10000_Audru_alajaam/RConn3 -- bus157/LConn1
  T_35394600_110000;35000;10000_Otepää_alajaam/RConn1 -- L_35394600/LConn1
  T_35394600_110000;35000;10000_Otepää_alajaam/RConn2 -- L_35394600/LConn2
  L_35394600/LConn3 -- T_35394600_110000;35000;10000_Otepää_alajaam/RConn3 -- bus158/LConn1
  T_35420119_110000;15000;400_Elva_alajaam/RConn1 -- L_35420119/LConn1
  T_35420119_110000;15000;400_Elva_alajaam/RConn2 -- L_35420119/LConn2
  L_35420119/LConn3 -- T_35420119_110000;15000;400_Elva_alajaam/RConn3 -- bus159/LConn1
  T_35367472_110000;35000;6000_Alutaguse_alajaam/RConn1 -- L_35367472/LConn1
  T_35367472_110000;35000;6000_Alutaguse_alajaam/RConn2 -- L_35367472/LConn2
  L_35367472/LConn3 -- T_35367472_110000;35000;6000_Alutaguse_alajaam/RConn3 -- bus160/LConn1
  T_35594689__/RConn1 -- L_35594689/LConn1
  T_35594689__/RConn2 -- L_35594689/LConn2
  L_35594689/LConn3 -- T_35594689__/RConn3 -- bus161/LConn1
  T_34903294_110000;35000;6000_Konsu_alajaam/RConn1 -- L_34903294/LConn1
  T_34903294_110000;35000;6000_Konsu_alajaam/RConn2 -- L_34903294/LConn2
  L_34903294/LConn3 -- T_34903294_110000;35000;6000_Konsu_alajaam/RConn3 -- bus162/LConn1
  T_263282454_110000;6000_Kiikla_alajaam/RConn1 -- L_263282454/LConn1
  T_263282454_110000;6000_Kiikla_alajaam/RConn2 -- L_263282454/LConn2
  L_263282454/LConn3 -- T_263282454_110000;6000_Kiikla_alajaam/RConn3 -- bus163/LConn1
  T_35367491_110000;35000;10000;6000_Aidu_alajaam/RConn1 -- L_35367491/LConn1
  T_35367491_110000;35000;10000;6000_Aidu_alajaam/RConn2 -- L_35367491/LConn2
  L_35367491/LConn3 -- T_35367491_110000;35000;10000;6000_Aidu_alajaam/RConn3 -- bus164/LConn1
  T_290177759_110000_Illuka_alajaam/RConn1 -- L_290177759/LConn1
  T_290177759_110000_Illuka_alajaam/RConn2 -- L_290177759/LConn2
  L_290177759/LConn3 -- T_290177759_110000_Illuka_alajaam/RConn3 -- bus165/LConn1
  T_35451776_110000;35000;15000;10000_Mustvee_alajaam/RConn1 -- L_35451776/LConn1
  T_35451776_110000;35000;15000;10000_Mustvee_alajaam/RConn2 -- L_35451776/LConn2
  L_35451776/LConn3 -- T_35451776_110000;35000;15000;10000_Mustvee_alajaam/RConn3 -- bus166/LConn1
  T_35451774_110000;35000;15000;10000_Jõgeva_alajaam/RConn1 -- L_35451774/LConn1
  T_35451774_110000;35000;15000;10000_Jõgeva_alajaam/RConn2 -- L_35451774/LConn2
  L_35451774/LConn3 -- T_35451774_110000;35000;15000;10000_Jõgeva_alajaam/RConn3 -- bus167/LConn1
  T_263282453_110000;10000_Kantküla_alajaam/RConn1 -- L_263282453/LConn1
  T_263282453_110000;10000_Kantküla_alajaam/RConn2 -- L_263282453/LConn2
  L_263282453/LConn3 -- T_263282453_110000;10000_Kantküla_alajaam/RConn3 -- bus168/LConn1
  T_35022089_110000;35000;10000_Sikassaare_alajaam/RConn1 -- L_35022089/LConn1
  T_35022089_110000;35000;10000_Sikassaare_alajaam/RConn2 -- L_35022089/LConn2
  L_35022089/LConn3 -- T_35022089_110000;35000;10000_Sikassaare_alajaam/RConn3 -- bus169/LConn1
  T_35022082_110000;10000_Orissaare_alajaam/RConn1 -- L_35022082/LConn1
  T_35022082_110000;10000_Orissaare_alajaam/RConn2 -- L_35022082/LConn2
  L_35022082/LConn3 -- T_35022082_110000;10000_Orissaare_alajaam/RConn3 -- bus170/LConn1
  T_35022087_110000;10000_Valjala_alajaam/RConn1 -- L_35022087/LConn1
  T_35022087_110000;10000_Valjala_alajaam/RConn2 -- L_35022087/LConn2
  L_35022087/LConn3 -- T_35022087_110000;10000_Valjala_alajaam/RConn3 -- bus171/LConn1
  T_35022100_110000;35000;10000_Leisi_alajaam/RConn1 -- L_35022100/LConn1
  T_35022100_110000;35000;10000_Leisi_alajaam/RConn2 -- L_35022100/LConn2
  L_35022100/LConn3 -- T_35022100_110000;35000;10000_Leisi_alajaam/RConn3 -- bus172/LConn1
  T_35367481_110000_Allika_alajaam/RConn1 -- L_35367481/LConn1
  T_35367481_110000_Allika_alajaam/RConn2 -- L_35367481/LConn2
  L_35367481/LConn3 -- T_35367481_110000_Allika_alajaam/RConn3 -- bus173/LConn1
  T_35451772_110000;15000_Suure_Jaani_alajaam/RConn1 -- L_35451772/LConn1
  T_35451772_110000;15000_Suure_Jaani_alajaam/RConn2 -- L_35451772/LConn2
  L_35451772/LConn3 -- T_35451772_110000;15000_Suure_Jaani_alajaam/RConn3 -- bus174/LConn1
  T_35451763_110000;35000;10000_Türi_alajaam/RConn1 -- L_35451763/LConn1
  T_35451763_110000;35000;10000_Türi_alajaam/RConn2 -- L_35451763/LConn2
  L_35451763/LConn3 -- T_35451763_110000;35000;10000_Türi_alajaam/RConn3 -- bus175/LConn1
  T_35594719__/RConn1 -- L_35594719/LConn1
  T_35594719__/RConn2 -- L_35594719/LConn2
  L_35594719/LConn3 -- T_35594719__/RConn3 -- bus176/LConn1
  T_34920713_110000;35000;10000_Väike_Maarja_alajaam/RConn1 -- L_34920713/LConn1
  T_34920713_110000;35000;10000_Väike_Maarja_alajaam/RConn2 -- L_34920713/LConn2
  L_34920713/LConn3 -- T_34920713_110000;35000;10000_Väike_Maarja_alajaam/RConn3 -- bus177/LConn1
  T_35445333__/RConn1 -- L_35445333/LConn1
  T_35445333__/RConn2 -- L_35445333/LConn2
  L_35445333/LConn3 -- T_35445333__/RConn3 -- bus178/LConn1
  T_35445334_110000;35000;10000_Võru_alajaam/RConn1 -- L_35445334/LConn1
  T_35445334_110000;35000;10000_Võru_alajaam/RConn2 -- L_35445334/LConn2
  L_35445334/LConn3 -- T_35445334_110000;35000;10000_Võru_alajaam/RConn3 -- bus179/LConn1
  T_35420117_110000;10000_Maaritsa_alajaam/RConn1 -- L_35420117/LConn1
  T_35420117_110000;10000_Maaritsa_alajaam/RConn2 -- L_35420117/LConn2
  L_35420117/LConn3 -- T_35420117_110000;10000_Maaritsa_alajaam/RConn3 -- bus180/LConn1
  T_262457166_110000;35000;15000;10000_Rõngu_alajaam/RConn1 -- L_262457166/LConn1
  T_262457166_110000;35000;15000;10000_Rõngu_alajaam/RConn2 -- L_262457166/LConn2
  L_262457166/LConn3 -- T_262457166_110000;35000;15000;10000_Rõngu_alajaam/RConn3 -- bus181/LConn1
  T_35445340_110000;10000_Soo_alajaam/RConn1 -- L_35445340/LConn1
  T_35445340_110000;10000_Soo_alajaam/RConn2 -- L_35445340/LConn2
  L_35445340/LConn3 -- T_35445340_110000;10000_Soo_alajaam/RConn3 -- bus182/LConn1
  T_35594687_110000;10000_Ruusa_alajaam/RConn1 -- L_35594687/LConn1
  T_35594687_110000;10000_Ruusa_alajaam/RConn2 -- L_35594687/LConn2
  L_35594687/LConn3 -- T_35594687_110000;10000_Ruusa_alajaam/RConn3 -- bus183/LConn1
  T_35445343__Põlva_alajaam/RConn1 -- L_35445343/LConn1
  T_35445343__Põlva_alajaam/RConn2 -- L_35445343/LConn2
  L_35445343/LConn3 -- T_35445343__Põlva_alajaam/RConn3 -- bus184/LConn1
  T_182242759_110000;10000_Rõuge_alajaam/RConn1 -- L_182242759/LConn1
  T_182242759_110000;10000_Rõuge_alajaam/RConn2 -- L_182242759/LConn2
  L_182242759/LConn3 -- T_182242759_110000;10000_Rõuge_alajaam/RConn3 -- bus185/LConn1
  T_35445335_110000;35000;10000_Mõniste_alajaam/RConn1 -- L_35445335/LConn1
  T_35445335_110000;35000;10000_Mõniste_alajaam/RConn2 -- L_35445335/LConn2
  L_35445335/LConn3 -- T_35445335_110000;35000;10000_Mõniste_alajaam/RConn3 -- bus186/LConn1
  T_182774903_110000;10000_Linda_alajaam/RConn1 -- L_182774903/LConn1
  T_182774903_110000;10000_Linda_alajaam/RConn2 -- L_182774903/LConn2
  L_182774903/LConn3 -- T_182774903_110000;10000_Linda_alajaam/RConn3 -- bus187/LConn1
  T_263235177_110000;10000_Sõmerpalu_alajaam/RConn1 -- L_263235177/LConn1
  T_263235177_110000;10000_Sõmerpalu_alajaam/RConn2 -- L_263235177/LConn2
  L_263235177/LConn3 -- T_263235177_110000;10000_Sõmerpalu_alajaam/RConn3 -- bus188/LConn1
  T_35445346_110000;10000_Kuuste_alajaam/RConn1 -- L_35445346/LConn1
  T_35445346_110000;10000_Kuuste_alajaam/RConn2 -- L_35445346/LConn2
  L_35445346/LConn3 -- T_35445346_110000;10000_Kuuste_alajaam/RConn3 -- bus189/LConn1
  T_30228363_110000;35000;15000;10000_Anne_alajaam/RConn1 -- L_30228363/LConn1
  T_30228363_110000;35000;15000;10000_Anne_alajaam/RConn2 -- L_30228363/LConn2
  L_30228363/LConn3 -- T_30228363_110000;35000;15000;10000_Anne_alajaam/RConn3 -- bus190/LConn1
  T_35594688_110000;15000_Alatskivi_alajaam/RConn1 -- L_35594688/LConn1
  T_35594688_110000;15000_Alatskivi_alajaam/RConn2 -- L_35594688/LConn2
  L_35594688/LConn3 -- T_35594688_110000;15000_Alatskivi_alajaam/RConn3 -- bus191/LConn1
  T_35445348_110000;15000_Tõrva_alajaam/RConn1 -- L_35445348/LConn1
  T_35445348_110000;15000_Tõrva_alajaam/RConn2 -- L_35445348/LConn2
  L_35445348/LConn3 -- T_35445348_110000;15000_Tõrva_alajaam/RConn3 -- bus192/LConn1
  T_35450872_110000;15000_Abja_alajaam/RConn1 -- L_35450872/LConn1
  T_35450872_110000;15000_Abja_alajaam/RConn2 -- L_35450872/LConn2
  L_35450872/LConn3 -- T_35450872_110000;15000_Abja_alajaam/RConn3 -- bus193/LConn1
  T_35450869_110000;10000_Valga_alajaam/RConn1 -- L_35450869/LConn1
  T_35450869_110000;10000_Valga_alajaam/RConn2 -- L_35450869/LConn2
  L_35450869/LConn3 -- T_35450869_110000;10000_Valga_alajaam/RConn3 -- bus194/LConn1
  T_262229346_110000;35000;10000_Keila_alajaam/RConn1 -- L_262229346/LConn1
  T_262229346_110000;35000;10000_Keila_alajaam/RConn2 -- L_262229346/LConn2
  L_262229346/LConn3 -- T_262229346_110000;35000;10000_Keila_alajaam/RConn3 -- bus195/LConn1
  T_34968246_110000;10000;6000_Järve_alajaam/RConn1 -- L_34968246/LConn1
  T_34968246_110000;10000;6000_Järve_alajaam/RConn2 -- L_34968246/LConn2
  L_34968246/LConn3 -- T_34968246_110000;10000;6000_Järve_alajaam/RConn3 -- bus196/LConn1
  T_34968285_110000;10000_Jüri_alajaam/RConn1 -- L_34968285/LConn1
  T_34968285_110000;10000_Jüri_alajaam/RConn2 -- L_34968285/LConn2
  L_34968285/LConn3 -- T_34968285_110000;10000_Jüri_alajaam/RConn3 -- bus197/LConn1
  T_35379710_110000;10000_Kohila_alajaam/RConn1 -- L_35379710/LConn1
  T_35379710_110000;10000_Kohila_alajaam/RConn2 -- L_35379710/LConn2
  L_35379710/LConn3 -- T_35379710_110000;10000_Kohila_alajaam/RConn3 -- bus198/LConn1
  T_34988535_110000;35000;10000;6000_Ellamaa_alajaam/RConn1 -- L_34988535/LConn1
  T_34988535_110000;35000;10000;6000_Ellamaa_alajaam/RConn2 -- L_34988535/LConn2
  L_34988535/LConn3 -- T_34988535_110000;35000;10000;6000_Ellamaa_alajaam/RConn3 -- bus199/LConn1
  T_34988502_110000;35000;10000_Risti_alajaam/RConn1 -- L_34988502/LConn1
  T_34988502_110000;35000;10000_Risti_alajaam/RConn2 -- L_34988502/LConn2
  L_34988502/LConn3 -- T_34988502_110000;35000;10000_Risti_alajaam/RConn3 -- bus200/LConn1
  T_34988471_110000;10000_Topi_alajaam/RConn1 -- L_34988471/LConn1
  T_34988471_110000;10000_Topi_alajaam/RConn2 -- L_34988471/LConn2
  L_34988471/LConn3 -- T_34988471_110000;10000_Topi_alajaam/RConn3 -- bus201/LConn1
  T_34935452_110000;35000;10000_Laagri_alajaam/RConn1 -- L_34935452/LConn1
  T_34935452_110000;35000;10000_Laagri_alajaam/RConn2 -- L_34935452/LConn2
  L_34935452/LConn3 -- T_34935452_110000;35000;10000_Laagri_alajaam/RConn3 -- bus202/LConn1
  T_34920702_110000;35000;10000_Rakvere_Põhja_alajaam/RConn1 -- L_34920702/LConn1
  T_34920702_110000;35000;10000_Rakvere_Põhja_alajaam/RConn2 -- L_34920702/LConn2
  L_34920702/LConn3 -- T_34920702_110000;35000;10000_Rakvere_Põhja_alajaam/RConn3 -- bus203/LConn1
  T_29595798_110000;35000;10000_Loo_alajaam/RConn1 -- L_29595798/LConn1
  T_29595798_110000;35000;10000_Loo_alajaam/RConn2 -- L_29595798/LConn2
  L_29595798/LConn3 -- T_29595798_110000;35000;10000_Loo_alajaam/RConn3 -- bus204/LConn1
  T_99350295_110000;35000;10000;6000_Veskimetsa_alajaam/RConn1 -- L_99350295/LConn1
  T_99350295_110000;35000;10000;6000_Veskimetsa_alajaam/RConn2 -- L_99350295/LConn2
  L_99350295/LConn3 -- T_99350295_110000;35000;10000;6000_Veskimetsa_alajaam/RConn3 -- bus205/LConn1
  T_99369449__Kadaka_alajaam/RConn1 -- L_99369449/LConn1
  T_99369449__Kadaka_alajaam/RConn2 -- L_99369449/LConn2
  L_99369449/LConn3 -- T_99369449__Kadaka_alajaam/RConn3 -- bus206/LConn1
  T_34988480_110000;10000_Tabasalu_alajaam/RConn1 -- L_34988480/LConn1
  T_34988480_110000;10000_Tabasalu_alajaam/RConn2 -- L_34988480/LConn2
  L_34988480/LConn3 -- T_34988480_110000;10000_Tabasalu_alajaam/RConn3 -- bus207/LConn1
  T_34968238_110000;35000;6000_Kopli_alajaam/RConn1 -- L_34968238/LConn1
  T_34968238_110000;35000;6000_Kopli_alajaam/RConn2 -- L_34968238/LConn2
  L_34968238/LConn3 -- T_34968238_110000;35000;6000_Kopli_alajaam/RConn3 -- bus208/LConn1
  T_34968239_110000;6000_Paljassaare_alajaam/RConn1 -- L_34968239/LConn1
  T_34968239_110000;6000_Paljassaare_alajaam/RConn2 -- L_34968239/LConn2
  L_34968239/LConn3 -- T_34968239_110000;6000_Paljassaare_alajaam/RConn3 -- bus209/LConn1
  T_85487602_110000;6000_Uus_Volta_alajaam/RConn1 -- L_85487602/LConn1
  T_85487602_110000;6000_Uus_Volta_alajaam/RConn2 -- L_85487602/LConn2
  L_85487602/LConn3 -- T_85487602_110000;6000_Uus_Volta_alajaam/RConn3 -- bus210/LConn1
  T_34968248_110000;35000;6000_Ülemiste_alajaam/RConn1 -- L_34968248/LConn1
  T_34968248_110000;35000;6000_Ülemiste_alajaam/RConn2 -- L_34968248/LConn2
  L_34968248/LConn3 -- T_34968248_110000;35000;6000_Ülemiste_alajaam/RConn3 -- bus211/LConn1
  T_34968251_110000;20000_Järveküla_alajaam/RConn1 -- L_34968251/LConn1
  T_34968251_110000;20000_Järveküla_alajaam/RConn2 -- L_34968251/LConn2
  L_34968251/LConn3 -- T_34968251_110000;20000_Järveküla_alajaam/RConn3 -- bus212/LConn1
  T_72668114_110000;10000_Iru_alajaam/RConn1 -- L_72668114/LConn1
  T_72668114_110000;10000_Iru_alajaam/RConn2 -- L_72668114/LConn2
  L_72668114/LConn3 -- T_72668114_110000;10000_Iru_alajaam/RConn3 -- bus213/LConn1
  T_34968269_110000;10000;6000_Lasnamäe_alajaam/RConn1 -- L_34968269/LConn1
  T_34968269_110000;10000;6000_Lasnamäe_alajaam/RConn2 -- L_34968269/LConn2
  L_34968269/LConn3 -- T_34968269_110000;10000;6000_Lasnamäe_alajaam/RConn3 -- bus214/LConn1
  T_35550404_110000;35000;10000_Paldiski_alajaam/RConn1 -- L_35550404/LConn1
  T_35550404_110000;35000;10000_Paldiski_alajaam/RConn2 -- L_35550404/LConn2
  L_35550404/LConn3 -- T_35550404_110000;35000;10000_Paldiski_alajaam/RConn3 -- bus215/LConn1
  T_35550410_110000;10000_Järvakandi_alajaam/RConn1 -- L_35550410/LConn1
  T_35550410_110000;10000_Järvakandi_alajaam/RConn2 -- L_35550410/LConn2
  L_35550410/LConn3 -- T_35550410_110000;10000_Järvakandi_alajaam/RConn3 -- bus216/LConn1
  T_35550412_110000;10000_Valgu_alajaam/RConn1 -- L_35550412/LConn1
  T_35550412_110000;10000_Valgu_alajaam/RConn2 -- L_35550412/LConn2
  L_35550412/LConn3 -- T_35550412_110000;10000_Valgu_alajaam/RConn3 -- bus217/LConn1
  T_35550415_110000;10000_Kehtna_alajaam/RConn1 -- L_35550415/LConn1
  T_35550415_110000;10000_Kehtna_alajaam/RConn2 -- L_35550415/LConn2
  L_35550415/LConn3 -- T_35550415_110000;10000_Kehtna_alajaam/RConn3 -- bus218/LConn1
  T_321829090_110000;10000_Joala_alajaam/RConn1 -- L_321829090/LConn1
  T_321829090_110000;10000_Joala_alajaam/RConn2 -- L_321829090/LConn2
  L_321829090/LConn3 -- T_321829090_110000;10000_Joala_alajaam/RConn3 -- bus219/LConn1
  T_94121285_110000_Kreenholmi_alajaam/RConn1 -- L_94121285/LConn1
  T_94121285_110000_Kreenholmi_alajaam/RConn2 -- L_94121285/LConn2
  L_94121285/LConn3 -- T_94121285_110000_Kreenholmi_alajaam/RConn3 -- bus220/LConn1
  T_35594708_110000;35000;6000_Narva_Peaalajaam/RConn1 -- L_35594708/LConn1
  T_35594708_110000;35000;6000_Narva_Peaalajaam/RConn2 -- L_35594708/LConn2
  L_35594708/LConn3 -- T_35594708_110000;35000;6000_Narva_Peaalajaam/RConn3 -- bus221/LConn1
  T_262755193_110000;10000_Vigala_alajaam/RConn1 -- L_262755193/LConn1
  T_262755193_110000;10000_Vigala_alajaam/RConn2 -- L_262755193/LConn2
  L_262755193/LConn3 -- T_262755193_110000;10000_Vigala_alajaam/RConn3 -- bus222/LConn1
  T_34968270_110000;10000_Ida_alajaam/RConn1 -- L_34968270/LConn1
  T_34968270_110000;10000_Ida_alajaam/RConn2 -- L_34968270/LConn2
  L_34968270/LConn3 -- T_34968270_110000;10000_Ida_alajaam/RConn3 -- bus223/LConn1
  T_34968274_110000;10000_Viimsi_alajaam/RConn1 -- L_34968274/LConn1
  T_34968274_110000;10000_Viimsi_alajaam/RConn2 -- L_34968274/LConn2
  L_34968274/LConn3 -- T_34968274_110000;10000_Viimsi_alajaam/RConn3 -- bus224/LConn1
  T_29979106_110000;35000;10000_Kallavere_alajaam/RConn1 -- L_29979106/LConn1
  T_29979106_110000;35000;10000_Kallavere_alajaam/RConn2 -- L_29979106/LConn2
  L_29979106/LConn3 -- T_29979106_110000;35000;10000_Kallavere_alajaam/RConn3 -- bus225/LConn1
  T_34968276_110000_Sadama_alajaam/RConn1 -- L_34968276/LConn1
  T_34968276_110000_Sadama_alajaam/RConn2 -- L_34968276/LConn2
  L_34968276/LConn3 -- T_34968276_110000_Sadama_alajaam/RConn3 -- bus226/LConn1
  T_101153487_110000;15000_Voldi_alajaam/RConn1 -- L_101153487/LConn1
  T_101153487_110000;15000_Voldi_alajaam/RConn2 -- L_101153487/LConn2
  L_101153487/LConn3 -- T_101153487_110000;15000_Voldi_alajaam/RConn3 -- bus227/LConn1
  T_35594741_110000;15000;6000;400_Puhja_alajaam/RConn1 -- L_35594741/LConn1
  T_35594741_110000;15000;6000;400_Puhja_alajaam/RConn2 -- L_35594741/LConn2
  L_35594741/LConn3 -- T_35594741_110000;15000;6000;400_Puhja_alajaam/RConn3 -- bus228/LConn1
  T_35555176__/RConn1 -- L_35555176/LConn1
  T_35555176__/RConn2 -- L_35555176/LConn2
  L_35555176/LConn3 -- T_35555176__/RConn3 -- bus229/LConn1
  T_34920683_110000;10000_Aseri_alajaam/RConn1 -- L_34920683/LConn1
  T_34920683_110000;10000_Aseri_alajaam/RConn2 -- L_34920683/LConn2
  L_34920683/LConn3 -- T_34920683_110000;10000_Aseri_alajaam/RConn3 -- bus230/LConn1
  T_34903268_110000;15000_Imavere_alajaam/RConn1 -- L_34903268/LConn1
  T_34903268_110000;15000_Imavere_alajaam/RConn2 -- L_34903268/LConn2
  L_34903268/LConn3 -- T_34903268_110000;15000_Imavere_alajaam/RConn3 -- bus231/LConn1
  T_35343350_110000;35000;10000_Aravete_alajaam/RConn1 -- L_35343350/LConn1
  T_35343350_110000;35000;10000_Aravete_alajaam/RConn2 -- L_35343350/LConn2
  L_35343350/LConn3 -- T_35343350_110000;35000;10000_Aravete_alajaam/RConn3 -- bus232/LConn1
  T_35343349__Roosna_Alliku_alajaam/RConn1 -- L_35343349/LConn1
  T_35343349__Roosna_Alliku_alajaam/RConn2 -- L_35343349/LConn2
  L_35343349/LConn3 -- T_35343349__Roosna_Alliku_alajaam/RConn3 -- bus233/LConn1
  T_35343353_110000;10000_Koigi_alajaam/RConn1 -- L_35343353/LConn1
  T_35343353_110000;10000_Koigi_alajaam/RConn2 -- L_35343353/LConn2
  L_35343353/LConn3 -- T_35343353_110000;10000_Koigi_alajaam/RConn3 -- bus234/LConn1
  T_34882447_110000;35000;15000;10000_Põltsamaa_alajaam/RConn1 -- L_34882447/LConn1
  T_34882447_110000;35000;15000;10000_Põltsamaa_alajaam/RConn2 -- L_34882447/LConn2
  L_34882447/LConn3 -- T_34882447_110000;35000;15000;10000_Põltsamaa_alajaam/RConn3 -- bus235/LConn1
  T_30222062_110000;10000_Emajõe_alajaam/RConn1 -- L_30222062/LConn1
  T_30222062_110000;10000_Emajõe_alajaam/RConn2 -- L_30222062/LConn2
  L_30222062/LConn3 -- T_30222062_110000;10000_Emajõe_alajaam/RConn3 -- bus236/LConn1
  T_35555175_110000;20000;10000;6000_Kunda_alajaam/RConn1 -- L_35555175/LConn1
  T_35555175_110000;20000;10000;6000_Kunda_alajaam/RConn2 -- L_35555175/LConn2
  L_35555175/LConn3 -- T_35555175_110000;20000;10000;6000_Kunda_alajaam/RConn3 -- bus237/LConn1
  T_35555173_110000_Viru_Nigula_alajaam/RConn1 -- L_35555173/LConn1
  T_35555173_110000_Viru_Nigula_alajaam/RConn2 -- L_35555173/LConn2
  L_35555173/LConn3 -- T_35555173_110000_Viru_Nigula_alajaam/RConn3 -- bus238/LConn1
  T_34920691_110000;35000;10000_Haljala_alajaam/RConn1 -- L_34920691/LConn1
  T_34920691_110000;35000;10000_Haljala_alajaam/RConn2 -- L_34920691/LConn2
  L_34920691/LConn3 -- T_34920691_110000;35000;10000_Haljala_alajaam/RConn3 -- bus239/LConn1
  T_35555163_110000;10000_Viitna_alajaam/RConn1 -- L_35555163/LConn1
  T_35555163_110000;10000_Viitna_alajaam/RConn2 -- L_35555163/LConn2
  L_35555163/LConn3 -- T_35555163_110000;10000_Viitna_alajaam/RConn3 -- bus240/LConn1
  T_35555166_110000;10000_Loksa_alajaam/RConn1 -- L_35555166/LConn1
  T_35555166_110000;10000_Loksa_alajaam/RConn2 -- L_35555166/LConn2
  L_35555166/LConn3 -- T_35555166_110000;10000_Loksa_alajaam/RConn3 -- bus241/LConn1
  T_35555165_110000;10000_Võsu_alajaam/RConn1 -- L_35555165/LConn1
  T_35555165_110000;10000_Võsu_alajaam/RConn2 -- L_35555165/LConn2
  L_35555165/LConn3 -- T_35555165_110000;10000_Võsu_alajaam/RConn3 -- bus242/LConn1
  T_35555161_110000;10000_Kadrina_alajaam/RConn1 -- L_35555161/LConn1
  T_35555161_110000;10000_Kadrina_alajaam/RConn2 -- L_35555161/LConn2
  L_35555161/LConn3 -- T_35555161_110000;10000_Kadrina_alajaam/RConn3 -- bus243/LConn1
  T_36977398_110000;15000_Oiu_alajaam/RConn1 -- L_36977398/LConn1
  T_36977398_110000;15000_Oiu_alajaam/RConn2 -- L_36977398/LConn2
  L_36977398/LConn3 -- T_36977398_110000;15000_Oiu_alajaam/RConn3 -- bus244/LConn1
  T_180118919_110000;15000;10000_Saare_alajaam/RConn1 -- L_180118919/LConn1
  T_180118919_110000;15000;10000_Saare_alajaam/RConn2 -- L_180118919/LConn2
  L_180118919/LConn3 -- T_180118919_110000;15000;10000_Saare_alajaam/RConn3 -- bus245/LConn1
  T_263253461_110000;10000_Ruusmäe_alajaam/RConn1 -- L_263253461/LConn1
  T_263253461_110000;10000_Ruusmäe_alajaam/RConn2 -- L_263253461/LConn2
  L_263253461/LConn3 -- T_263253461_110000;10000_Ruusmäe_alajaam/RConn3 -- bus246/LConn1
  T_35022081_110000;10000_Muhu_alajaam/RConn1 -- L_35022081/LConn1
  T_35022081_110000;10000_Muhu_alajaam/RConn2 -- L_35022081/LConn2
  L_35022081/LConn3 -- T_35022081_110000;10000_Muhu_alajaam/RConn3 -- bus247/LConn1
  T_34988518_110000;35000;10000_Võiküla_alajaam/RConn1 -- L_34988518/LConn1
  T_34988518_110000;35000;10000_Võiküla_alajaam/RConn2 -- L_34988518/LConn2
  L_34988518/LConn3 -- T_34988518_110000;35000;10000_Võiküla_alajaam/RConn3 -- bus248/LConn1
  T_34988522_110000;35000;10000_Tusti_alajaam/RConn1 -- L_34988522/LConn1
  T_34988522_110000;35000;10000_Tusti_alajaam/RConn2 -- L_34988522/LConn2
  L_34988522/LConn3 -- T_34988522_110000;35000;10000_Tusti_alajaam/RConn3 -- bus249/LConn1
  T_29978896_110000;20000_Jägala_alajaam/RConn1 -- L_29978896/LConn1
  T_29978896_110000;20000_Jägala_alajaam/RConn2 -- L_29978896/LConn2
  L_29978896/LConn3 -- T_29978896_110000;20000_Jägala_alajaam/RConn3 -- bus250/LConn1
  T_35384083_110000;35000;10000_Kuusalu_alajaam/RConn1 -- L_35384083/LConn1
  T_35384083_110000;35000;10000_Kuusalu_alajaam/RConn2 -- L_35384083/LConn2
  L_35384083/LConn3 -- T_35384083_110000;35000;10000_Kuusalu_alajaam/RConn3 -- bus251/LConn1
  T_35555171_110000;10000_Kolga_alajaam/RConn1 -- L_35555171/LConn1
  T_35555171_110000;10000_Kolga_alajaam/RConn2 -- L_35555171/LConn2
  L_35555171/LConn3 -- T_35555171_110000;10000_Kolga_alajaam/RConn3 -- bus252/LConn1
  T_263282458_110000;10000_Põdra_alajaam/RConn1 -- L_263282458/LConn1
  T_263282458_110000;10000_Põdra_alajaam/RConn2 -- L_263282458/LConn2
  L_263282458/LConn3 -- T_263282458_110000;10000_Põdra_alajaam/RConn3 -- bus253/LConn1
  T_34988486_110000;35000;10000_Rummu_alajaam/RConn1 -- L_34988486/LConn1
  T_34988486_110000;35000;10000_Rummu_alajaam/RConn2 -- L_34988486/LConn2
  L_34988486/LConn3 -- T_34988486_110000;35000;10000_Rummu_alajaam/RConn3 -- bus254/LConn1
  T_34988525_110000;10000_Martna_alajaam/RConn1 -- L_34988525/LConn1
  T_34988525_110000;10000_Martna_alajaam/RConn2 -- L_34988525/LConn2
  L_34988525/LConn3 -- T_34988525_110000;10000_Martna_alajaam/RConn3 -- bus255/LConn1
  T_35594731_110000;10000_Kullamaa_alajaam/RConn1 -- L_35594731/LConn1
  T_35594731_110000;10000_Kullamaa_alajaam/RConn2 -- L_35594731/LConn2
  L_35594731/LConn3 -- T_35594731_110000;10000_Kullamaa_alajaam/RConn3 -- bus256/LConn1
  T_101177924_110000_Aulepa_alajaam/RConn1 -- L_101177924/LConn1
  T_101177924_110000_Aulepa_alajaam/RConn2 -- L_101177924/LConn2
  L_101177924/LConn3 -- T_101177924_110000_Aulepa_alajaam/RConn3 -- bus257/LConn1
  T_34988531_110000;10000_Taebla_alajaam/RConn1 -- L_34988531/LConn1
  T_34988531_110000;10000_Taebla_alajaam/RConn2 -- L_34988531/LConn2
  L_34988531/LConn3 -- T_34988531_110000;10000_Taebla_alajaam/RConn3 -- bus258/LConn1
  T_34988527_110000;35000;10000_Haapsalu_alajaam/RConn1 -- L_34988527/LConn1
  T_34988527_110000;35000;10000_Haapsalu_alajaam/RConn2 -- L_34988527/LConn2
  L_34988527/LConn3 -- T_34988527_110000;35000;10000_Haapsalu_alajaam/RConn3 -- bus259/LConn1
  T_34988495_110000;10000_Nõva_alajaam/RConn1 -- L_34988495/LConn1
  T_34988495_110000;10000_Nõva_alajaam/RConn2 -- L_34988495/LConn2
  L_34988495/LConn3 -- T_34988495_110000;10000_Nõva_alajaam/RConn3 -- bus260/LConn1
  T_34685101_330000_Eesti_EJ_alajaam/RConn1 -- L_34685101/LConn1
  T_34685101_330000_Eesti_EJ_alajaam/RConn2 -- L_34685101/LConn2
  L_34685101/LConn3 -- T_34685101_330000_Eesti_EJ_alajaam/RConn3 -- bus261/LConn1
